simulink library "ammclib_bam_S32K3xx"  (R2016a)
settings: Solver=VariableStepAuto  SolverMode=SingleTasking  StartTime=0.0  StopTime=10.0  RelTol=1e-3
undefined symbols (not defined in the file or in its folder): a1, a2, ADCMaxError, autoCalcEn, b0, b1, b2, cfg, dgain, escale, f16A1, f16A2, f16ADCMaxError, f16B0, f16B1, f16B2, f16C1, f16CC1sc, f16CC1sc_D, f16CC1sc_Q, f16CC2sc, f16CC2sc_D, f16CC2sc_Q, f16DerivGain, f16EGain, f16FiltCoef, f16HystOff, f16HystOn, f16IGain, f16IntegGain, f16IntegGain_D, f16IntegGain_Q, f16IntegGainQ, f16Kd, f16KLs, f16Kq, f16KRs, f16Limit, f16LowerLimit, f16LowerLimit_D, f16LowerLimit_Q, f16LowerLimitQ, f16ModIndex, f16OutValOff, f16OutValOn, f16PropGain, f16PropGain_D, f16PropGain_Q, f16PropGainQ, f16RampDown, f16RampUp, f16UGain, f16UpperLimit, f16UpperLimit_D, f16UpperLimit_Q, f16UpperLimitQ, f16WIGain, f32A1, f32A2, f32ADCMaxError ... (+180)
(part 39 of 50)

== system ammclib_bam_S32K3xx/GFLIB/FLT ==
  GFLIB_Acos_FLT : Subsystem  TreatAsAtomicUnit=on  mask(GFLIB_Acos_FLT){}
      mask help: Inverse cosine function in single precision floating-point implementation. Refer to the AMMCLIB User's Guide for further details.
      mask init: same as ammclib_bam_S32K3xx/GDFLIB/F16/GDFLIB_FilterFIR_F16
      settings: RTWSystemCode=Inline
      mask Help: web([fileparts(which('ammclib_bam_S32K3xx.slx')) '/../doc/S32K3XXMCLUG.pdf'], '-browser')
      mask Display: pos = get_param(gcb, 'Position');width = pos(3) - pos(1); height = pos(4) - pos(2);tX=width/2;tY=height - 8;color('black');text(tX,tY, 'GFLIB_Acos_FLT', 'horizontalAlignment', 'center');
  GFLIB_Asin_FLT : Subsystem  TreatAsAtomicUnit=on  mask(GFLIB_Asin_FLT){}
      mask help: Inverse sine function in single precision floating-point implementation. Refer to the AMMCLIB User's Guide for further details.
      mask init: same as ammclib_bam_S32K3xx/GDFLIB/F16/GDFLIB_FilterFIR_F16
      settings: RTWSystemCode=Inline
      mask Help: web([fileparts(which('ammclib_bam_S32K3xx.slx')) '/../doc/S32K3XXMCLUG.pdf'], '-browser')
      mask Display: pos = get_param(gcb, 'Position');width = pos(3) - pos(1); height = pos(4) - pos(2);tX=width/2;tY=height - 8;color('black');text(tX,tY, 'GFLIB_Asin_FLT', 'horizontalAlignment', 'center');
  GFLIB_AtanYXShifted_FLT : Subsystem  TreatAsAtomicUnit=on  mask(GFLIB_AtanYXShifted_FLT){}
      mask help: Shifted arctangent of two arguments Y/X in single precision floating-point implementation. Refer to the AMMCLIB User's Guide for further details.
      mask init: same as ammclib_bam_S32K3xx/GDFLIB/F16/GDFLIB_FilterFIR_F16
      settings: RTWSystemCode=Inline
      mask Help: web([fileparts(which('ammclib_bam_S32K3xx.slx')) '/../doc/S32K3XXMCLUG.pdf'], '-browser')
      mask Display: pos = get_param(gcb, 'Position');width = pos(3) - pos(1); height = pos(4) - pos(2);tX=width/2;tY=height - 8;color('black');text(tX,tY, 'GFLIB_AtanYXShifted_FLT', 'horizontalAlignment', 'center');
  GFLIB_AtanYX_FLT : Subsystem  TreatAsAtomicUnit=on  mask(GFLIB_AtanYX_FLT){}
      mask help: Arctangent of two arguments Y/X in single precision floating-point implementation. Refer to the AMMCLIB User's Guide for further details.
      mask init: same as ammclib_bam_S32K3xx/GDFLIB/F16/GDFLIB_FilterFIR_F16
      settings: RTWSystemCode=Inline
      mask Help: web([fileparts(which('ammclib_bam_S32K3xx.slx')) '/../doc/S32K3XXMCLUG.pdf'], '-browser')
      mask Display: pos = get_param(gcb, 'Position');width = pos(3) - pos(1); height = pos(4) - pos(2);tX=width/2;tY=height - 8;color('black');text(tX,tY, 'GFLIB_AtanYX_FLT', 'horizontalAlignment', 'center');
  GFLIB_Atan_FLT : Subsystem  TreatAsAtomicUnit=on  mask(GFLIB_Atan_FLT){}
      mask help: Inverse tangent function in single precision floating-point implementation. Refer to the AMMCLIB User's Guide for further details.
      mask init: same as ammclib_bam_S32K3xx/GDFLIB/F16/GDFLIB_FilterFIR_F16
      settings: RTWSystemCode=Inline
      mask Help: web([fileparts(which('ammclib_bam_S32K3xx.slx')) '/../doc/S32K3XXMCLUG.pdf'], '-browser')
      mask Display: pos = get_param(gcb, 'Position');width = pos(3) - pos(1); height = pos(4) - pos(2);tX=width/2;tY=height - 8;color('black');text(tX,tY, 'GFLIB_Atan_FLT', 'horizontalAlignment', 'center');
  GFLIB_ControllerPIDpAW_FLT : Subsystem  StartFcn=|  TreatAsAtomicUnit=on  mask(GFLIB_ControllerPIDpAW_FLT){showStates=Hide (faster execution), resetStatesEnable=Pre-set according to the first set of inputs after reset, SampleTime=-1, pgain=5, igain=0.5, dgain=0.01, filtCoef=10, lowerLimit=-10, upperLimit=10, autoCalcEn=on, fltPropGain=0, fltIntegGain=0, fltDerivGain=0, fltFiltCoef=0, fltLowerLimit=0, fltUpperLimit=0, SampleTime_1=NaN}
      | ts=get_param(gcb,'CompiledSampleTime');
      | if iscell(ts)
      |   ts=ts{1};
      |   if iscell(ts)
      |     ts=ts{1};
      |   end
      | end
      | ts=ts(1);
      | set_param(gcb,'SampleTime_1',num2str(ts));
      | p=Simulink.Mask.get(gcb);
      | hintText=p.getDialogControl('timeHint');
      | SampleTime=Simulink.data.evalinGlobal(bdroot,get_param(gcb,'SampleTime'));
      | p=Simulink.Mask.get(gcb);
      | autoCalcEn=get_param(gcb,'autoCalcEn');
      | if strcmp(autoCalcEn,'on')
      |   if SampleTime==-1
      |     hintText.Prompt='Caution: Implementation parameters depend on inherited sample time. Make sure that the sample time of the block''s inputs corresponds to the sampling period in the target application.';
      |   else
      |     hintText.Prompt='Caution: Implementation parameters depend on the sample time. Make sure that the simulation time step corresponds to the sampling period in the target application.';
      |   end
      |   SampleTime=ts;
      |   fltPropGain_bkup=get_param(gcb,'fltPropGain');
      |   fltIntegGain_bkup=get_param(gcb,'fltIntegGain');
      |   fltDerivGain_bkup=get_param(gcb,'fltDerivGain');
      |   fltFiltCoef_bkup=get_param(gcb,'fltFiltCoef');
      |   fltLowerLimit_bkup=get_param(gcb,'fltLowerLimit');
      |   fltUpperLimit_bkup=get_param(gcb,'fltUpperLimit');
      |   pgain=Simulink.data.evalinGlobal(bdroot,get_param(gcb,'pgain'));
      |   igain=Simulink.data.evalinGlobal(bdroot,get_param(gcb,'igain'));
      |   dgain=Simulink.data.evalinGlobal(bdroot,get_param(gcb,'dgain'));
      |   filtCoef=Simulink.data.evalinGlobal(bdroot,get_param(gcb,'filtCoef'));
      |   lowerLimit=Simulink.data.evalinGlobal(bdroot,get_param(gcb,'lowerLimit'));
      |   upperLimit=Simulink.data.evalinGlobal(bdroot,get_param(gcb,'upperLimit'));
      |   if (upperLimit<=lowerLimit)
      |     warning('UpperLimit should be greater than LowerLimit.');
      |   end
      |   fltPropGain=pgain;
      |   fltIntegGain=igain*SampleTime*0.5;
      |   exparg=-SampleTime*filtCoef;
      |   expconst=exp(exparg);
      |   fltFiltCoef=expconst;
      |   fltDerivGain=dgain/SampleTime*(1 - expconst);
      |   fltUpperLimit=upperLimit;
      |   fltLowerLimit=lowerLimit;
      |   if isnan(fltPropGain)
      |     if ~strcmp(fltPropGain_bkup,'0')
      |       set_param(gcb,'fltPropGain','0');
      |     end
      |   else
      |     tmps=num2str(fltPropGain);
      |     if ~strcmp(fltPropGain_bkup,tmps)
      |       set_param(gcb,'fltPropGain',tmps);
      |     end
      |   end
      |   if isnan(fltIntegGain)
      |     if ~strcmp(fltIntegGain_bkup,'0')
      |       set_param(gcb,'fltIntegGain','0');
      |     end
      |   else
      |     tmps=num2str(fltIntegGain);
      |     if ~strcmp(fltIntegGain_bkup,tmps)
      |       set_param(gcb,'fltIntegGain',tmps);
      |     end
      |   end
      |   if isnan(fltDerivGain)
      |     if ~strcmp(fltDerivGain_bkup,'0')
      |       set_param(gcb,'fltDerivGain','0');
      |     end
      |   else
      |     tmps=num2str(fltDerivGain);
      |     if ~strcmp(fltDerivGain_bkup,tmps)
      |       set_param(gcb,'fltDerivGain',tmps);
      |     end
      |   end
      |   if isnan(fltFiltCoef)
      |     if ~strcmp(fltFiltCoef_bkup,'0')
      |       set_param(gcb,'fltFiltCoef','0');
      |     end
      |   else
      |     tmps=num2str(fltFiltCoef);
      |     if ~strcmp(fltFiltCoef_bkup,tmps)
      |       set_param(gcb,'fltFiltCoef',tmps);
      |     end
      |   end
      |   if isnan(fltLowerLimit)
      |     if ~strcmp(fltLowerLimit_bkup,'0')
      |       set_param(gcb,'fltLowerLimit','0');
      |     end
      |   else
      |     tmps=num2str(fltLowerLimit);
      |     if ~strcmp(fltLowerLimit_bkup,tmps)
      |       set_param(gcb,'fltLowerLimit',tmps);
      |     end
      |   end
      |   if isnan(fltUpperLimit)
      |     if ~strcmp(fltUpperLimit_bkup,'0')
      |       set_param(gcb,'fltUpperLimit','0');
      |     end
      |   else
      |     tmps=num2str(fltUpperLimit);
      |     if ~strcmp(fltUpperLimit_bkup,tmps)
      |       set_param(gcb,'fltUpperLimit',tmps);
      |     end
      |   end
      | end
      mask prompts: showStates "Show internal states:"; resetStatesEnable "Internal state after reset:"; SampleTime "Sample time (-1 for inherited):"; pgain "Proportional gain (P):"; igain "Integral gain (I):"; dgain "Derivative gain (D):"; filtCoef "Derivative gain limit N (usually 3 to 20):"; lowerLimit "Controller lower limit:"; upperLimit "Controller upper limit:"; autoCalcEn "Calculate implementation parameters from physical parameters"; fltPropGain "fltPropGain (Proportional gain):"; fltIntegGain "fltIntegGain (Integral gain):"; fltDerivGain "fltDerivGain (Derivative Gain):"; fltFiltCoef "fltFiltCoef (Derivative term filter coefficient):"; fltLowerLimit "fltLowerLimit (Lower Limit of the controller):"; fltUpperLimit "fltUpperLimit (Upper Limit of the controller):"; SampleTime_1 "Discrete sample time:"
      mask help: Parallel form of a discrete-time PID controller with anti-windup in single precision floating-point implementation. This block supports re-initialization of the internal state during simulation. If the block is reset, the controller's output will be aligned with the input fltControllerPIDpAWOut_preset. Refer to the AMMCLIB User's Guide for further details.
      mask init:
      | ddName = get_param(bdroot,'DataDictionary');
      | if length(ddName)==0
      |   set_param(bdroot,'DataDictionary','ammclib_types.sldd');
      | else
      |   dd = Simulink.data.dictionary.open(ddName);
      |   data = getSection(dd,'Design Data');
      |   if ~exist(data,'SWLIBS_2Syst_F16')
      |     addDataSource(dd,'ammclib_types.sldd');
      |     saveChanges(dd);
      |   end
      | end
      | 
      | if showStates == 1
      |   % hidden state variables
      |   if strcmp(get_param([gcb '/fltPropGain'], 'BlockType'), 'Inport')
      |     posblk = get_param(gcb, 'Position');
      | 
      |     pos = get_param([gcb, '/fltPropGain'], 'Position');
      |     orient = get_param([gcb, '/fltPropGain'], 'Orientation');
      |     delete_block([gcb, '/fltPropGain']);
      |     add_block('built-in/Ground', [gcb, '/fltPropGain'], 'Position', pos, 'Orientation', orient);
      | 
      |     pos = get_param([gcb, '/fltIntegGain'], 'Position');
      |     orient = get_param([gcb, '/fltIntegGain'], 'Orientation');
      |     delete_block([gcb, '/fltIntegGain']);
      |     add_block('built-in/Ground', [gcb, '/fltIntegGain'], 'Position', pos, 'Orientation', orient);
      | 
      |     pos = get_param([gcb, '/fltDerivGain'], 'Position');
      |     orient = get_param([gcb, '/fltDerivGain'], 'Orientation');
      |     delete_block([gcb, '/fltDerivGain']);
      |     add_block('built-in/Ground', [gcb, '/fltDerivGain'], 'Position', pos, 'Orientation', orient);
      | 
      |     pos = get_param([gcb, '/fltFiltCoef'], 'Position');
      |     orient = get_param([gcb, '/fltFiltCoef'], 'Orientation');
      |     delete_block([gcb, '/fltFiltCoef']);
      |     add_block('built-in/Ground', [gcb, '/fltFiltCoef'], 'Position', pos, 'Orientation', orient);
      | 
      |     pos = get_param([gcb, '/fltLowerLimit'], 'Position');
      |     orient = get_param([gcb, '/fltLowerLimit'], 'Orientation');
      |     delete_block([gcb, '/fltLowerLimit']);
      |     add_block('built-in/Ground', [gcb, '/fltLowerLimit'], 'Position', pos, 'Orientation', orient);
      | 
      |     pos = get_param([gcb, '/fltUpperLimit'], 'Position');
      |     orient = get_param([gcb, '/fltUpperLimit'], 'Orientation');
      |     delete_block([gcb, '/fltUpperLimit']);
      |     add_block('built-in/Ground', [gcb, '/fltUpperLimit'], 'Position', pos, 'Orientation', orient);
      | 
      |     pos = get_param([gcb, '/fltIntegPartK_1'], 'Position');
      |     orient = get_param([gcb, '/fltIntegPartK_1'], 'Orientation');
      |     delete_block([gcb, '/fltIntegPartK_1']);
      |     add_block('built-in/Ground', [gcb, '/fltIntegPartK_1'], 'Position', pos, 'Orientation', orient);
      | 
      |     pos = get_param([gcb, '/fltDerivPartK_1'], 'Position');
      |     orient = get_param([gcb, '/fltDerivPartK_1'], 'Orientation');
      |     delete_block([gcb, '/fltDerivPartK_1']);
      |     add_block('built-in/Ground', [gcb, '/fltDerivPartK_1'], 'Position', pos, 'Orientation', orient);
      | 
      |     pos = get_param([gcb, '/fltInK_1'], 'Position');
      |     orient = get_param([gcb, '/fltInK_1'], 'Orientation');
      |     delete_block([gcb, '/fltInK_1']);
      |     add_block('built-in/Ground', [gcb, '/fltInK_1'], 'Position', pos, 'Orientation', orient);
      | 
      | 
      |     pmask=Simulink.Mask.get(gcb);
      |     pctrl=pmask.getParameter('SampleTime');
      |     pctrl.set('TypeOptions',{'fltInErr/SampleTime','fltControllerPIDpAWOut_preset/SampleTime'});
      | 
      |     pos = get_param([gcb '/fltIntegPartK_1_Out'], 'Position');
      |     orient = get_param([gcb '/fltIntegPartK_1_Out'], 'Orientation');
      |     delete_block([gcb '/fltIntegPartK_1_Out']);
      |     add_block('built-in/Terminator', [gcb '/fltIntegPartK_1_Out'], 'Position', pos, 'Orientation', orient);
      | 
      |     pos = get_param([gcb '/fltDerivPartK_1_Out'], 'Position');
      |     orient = get_param([gcb '/fltDerivPartK_1_Out'], 'Orientation');
      |     delete_block([gcb '/fltDerivPartK_1_Out']);
      |     add_block('built-in/Terminator', [gcb '/fltDerivPartK_1_Out'], 'Position', pos, 'Orientation', orient);
      | 
      |     pos = get_param([gcb '/fltInK_1_Out'], 'Position');
      |     orient = get_param([gcb '/fltInK_1_Out'], 'Orientation');
      |     delete_block([gcb '/fltInK_1_Out']);
      |     add_block('built-in/Terminator', [gcb '/fltInK_1_Out'], 'Position', pos, 'Orientation', orient);
      | 
      |     set_param([gcb '/fltInErr'], 'Port', '1');
      |     set_param([gcb '/fltControllerPIDpAWOut_preset'], 'Port', '2');
      | 
      |     tmpOutCnt=0;
      |     tmpOutCnt=tmpOutCnt+1;
      |     set_param([gcb '/fltOut'], 'Port', num2str(tmpOutCnt));
      |     tmpOutCnt=tmpOutCnt+1;
      |     set_param([gcb '/u16LimitFlag'], 'Port', num2str(tmpOutCnt));
      | 
      |     autoCalcEn=get_param(gcb,'autoCalcEn');
      |     if strcmp(autoCalcEn,'on')
      |       set_param(gcb,'MaskEnables',{'on','on','on','on','on','on','on','on','on','on','on','on','on','on','on','on','off'});
      |     else
      |       set_param(gcb,'MaskEnables',{'on','on','on','off','off','off','off','off','off','on','on','on','on','on','on','on','off'});
      |     end
      | 
      |     if (posblk(4) - posblk(2)) > 75
      |       height = 75;
      |       set_param(gcb,'Position',[posblk(1), posblk(2), posblk(3), posblk(2)+height])
      |     end
      |   end
      | else
      |   % shown state variables
      |   if strcmp(get_param([gcb '/fltPropGain'], 'BlockType'), 'Ground')
      |     posblk = get_param(gcb, 'Position');
      | 
      |     pos = get_param([gcb, '/fltPropGain'], 'Position');
      |     orient = get_param([gcb, '/fltPropGain'], 'Orientation');
      |     delete_block([gcb, '/fltPropGain']);
      |     add_block('built-in/Inport', [gcb, '/fltPropGain'], 'Position', pos, 'Orientation', orient, 'OutDataTypeStr', 'single');
      | 
      |     pos = get_param([gcb, '/fltIntegGain'], 'Position');
      |     orient = get_param([gcb, '/fltIntegGain'], 'Orientation');
      |     delete_block([gcb, '/fltIntegGain']);
      |     add_block('built-in/Inport', [gcb, '/fltIntegGain'], 'Position', pos, 'Orientation', orient, 'OutDataTypeStr', 'single');
      | 
      |     pos = get_param([gcb, '/fltDerivGain'], 'Position');
      |     orient = get_param([gcb, '/fltDerivGain'], 'Orientation');
      |     delete_block([gcb, '/fltDerivGain']);
      |     add_block('built-in/Inport', [gcb, '/fltDerivGain'], 'Position', pos, 'Orientation', orient, 'OutDataTypeStr', 'single');
      | 
      |     pos = get_param([gcb, '/fltFiltCoef'], 'Position');
      |     orient = get_param([gcb, '/fltFiltCoef'], 'Orientation');
      |     delete_block([gcb, '/fltFiltCoef']);
      |     add_block('built-in/Inport', [gcb, '/fltFiltCoef'], 'Position', pos, 'Orientation', orient, 'OutDataTypeStr', 'single');
      | 
      |     pos = get_param([gcb, '/fltLowerLimit'], 'Position');
      |     orient = get_param([gcb, '/fltLowerLimit'], 'Orientation');
      |     delete_block([gcb, '/fltLowerLimit']);
      |     add_block('built-in/Inport', [gcb, '/fltLowerLimit'], 'Position', pos, 'Orientation', orient, 'OutDataTypeStr', 'single');
      | 
      |     pos = get_param([gcb, '/fltUpperLimit'], 'Position');
      |     orient = get_param([gcb, '/fltUpperLimit'], 'Orientation');
      |     delete_block([gcb, '/fltUpperLimit']);
      |     add_block('built-in/Inport', [gcb, '/fltUpperLimit'], 'Position', pos, 'Orientation', orient, 'OutDataTypeStr', 'single');
      | 
      |     pos = get_param([gcb, '/fltIntegPartK_1'], 'Position');
      |     orient = get_param([gcb, '/fltIntegPartK_1'], 'Orientation');
      |     delete_block([gcb, '/fltIntegPartK_1']);
      |     add_block('built-in/Inport', [gcb, '/fltIntegPartK_1'], 'Position', pos, 'Orientation', orient, 'OutDataTypeStr', 'single');
      | 
      |     pos = get_param([gcb, '/fltDerivPartK_1'], 'Position');
      |     orient = get_param([gcb, '/fltDerivPartK_1'], 'Orientation');
      |     delete_block([gcb, '/fltDerivPartK_1']);
      |     add_block('built-in/Inport', [gcb, '/fltDerivPartK_1'], 'Position', pos, 'Orientation', orient, 'OutDataTypeStr', 'single');
      | 
      |     pos = get_param([gcb, '/fltInK_1'], 'Position');
      |     orient = get_param([gcb, '/fltInK_1'], 'Orientation');
      |     delete_block([gcb, '/fltInK_1']);
      |     add_block('built-in/Inport', [gcb, '/fltInK_1'], 'Position', pos, 'Orientation', orient, 'OutDataTypeStr', 'single');
      | 
      | 
      | 
      |     pos = get_param([gcb '/fltIntegPartK_1_Out'], 'Position');
      |     orient = get_param([gcb '/fltIntegPartK_1_Out'], 'Orientation');
      |     delete_block([gcb '/fltIntegPartK_1_Out']);
      |     add_block('built-in/Outport', [gcb '/fltIntegPartK_1_Out'], 'Position', pos, 'Orientation', orient);
      | 
      |     pos = get_param([gcb '/fltDerivPartK_1_Out'], 'Position');
      |     orient = get_param([gcb '/fltDerivPartK_1_Out'], 'Orientation');
      |     delete_block([gcb '/fltDerivPartK_1_Out']);
      |     add_block('built-in/Outport', [gcb '/fltDerivPartK_1_Out'], 'Position', pos, 'Orientation', orient);
      | 
      |     pos = get_param([gcb '/fltInK_1_Out'], 'Position');
      |     orient = get_param([gcb '/fltInK_1_Out'], 'Orientation');
      |     delete_block([gcb '/fltInK_1_Out']);
      |     add_block('built-in/Outport', [gcb '/fltInK_1_Out'], 'Position', pos, 'Orientation', orient);
      | 
      | 
      |     pmask=Simulink.Mask.get(gcb);
      |     pctrl=pmask.getParameter('SampleTime');
      |     pctrl.set('TypeOptions',{'fltInErr/SampleTime','fltControllerPIDpAWOut_preset/SampleTime','fltPropGain/SampleTime','fltIntegGain/SampleTime','fltDerivGain/SampleTime','fltFiltCoef/SampleTime','fltLowerLimit/SampleTime','fltUpperLimit/SampleTime','fltIntegPartK_1/SampleTime','fltDerivPartK_1/SampleTime','fltInK_1/SampleTime'});
      | 
      |     set_param([gcb '/fltInErr'], 'Port', '1');
      |     set_param([gcb '/fltControllerPIDpAWOut_preset'], 'Port', '2');
      |     set_param([gcb '/fltPropGain'], 'Port', '3');
      |     set_param([gcb '/fltIntegGain'], 'Port', '4');
      |     set_param([gcb '/fltDerivGain'], 'Port', '5');
      |     set_param([gcb '/fltFiltCoef'], 'Port', '6');
      |     set_param([gcb '/fltLowerLimit'], 'Port', '7');
      |     set_param([gcb '/fltUpperLimit'], 'Port', '8');
      |     set_param([gcb '/fltIntegPartK_1'], 'Port', '9');
      |     set_param([gcb '/fltDerivPartK_1'], 'Port', '10');
      |     set_param([gcb '/fltInK_1'], 'Port', '11');
      | 
      |     tmpOutCnt=0;
      |     tmpOutCnt=tmpOutCnt+1;
      |     set_param([gcb '/fltOut'], 'Port', num2str(tmpOutCnt));
      |     tmpOutCnt=tmpOutCnt+1;
      |     set_param([gcb '/u16LimitFlag'], 'Port', num2str(tmpOutCnt));
      |     tmpOutCnt=tmpOutCnt+1;
      |     set_param([gcb '/fltIntegPartK_1_Out'], 'Port', num2str(tmpOutCnt));
      |     tmpOutCnt=tmpOutCnt+1;
      |     set_param([gcb '/fltDerivPartK_1_Out'], 'Port', num2str(tmpOutCnt));
      |     tmpOutCnt=tmpOutCnt+1;
      |     set_param([gcb '/fltInK_1_Out'], 'Port', num2str(tmpOutCnt));
      | 
      |     set_param(gcb,'MaskEnables',{'on','on','on','off','off','off','off','off','off','off','off','off','off','off','off','off','off'});
      | 
      |     if (posblk(4) - posblk(2)) < 300
      |       height = 300;
      |       set_param(gcb,'Position',[posblk(1), posblk(2), posblk(3), posblk(2)+height])
      |     end
      |   end
      | end
      settings: RTWSystemCode=Inline
      mask Help: web([fileparts(which('ammclib_bam_S32K3xx.slx')) '/../doc/S32K3XXMCLUG.pdf'], '-browser')
      mask TypeOptions showStates: Hide (faster execution) | Show (allows debugging; connect feedback loops manually)
      mask Callback showStates:
      | maskStr=get_param(gcb,'showStates');
      | if strcmp(maskStr,'Hide (faster execution)')
      |   if strcmp(get_param([gcb '/fltPropGain'], 'BlockType'), 'Inport')
      |     autoCalcEn=get_param(gcb,'autoCalcEn');
      |     if strcmp(autoCalcEn,'on')
      |       set_param(gcb,'MaskEnables',{'on','on','on','on','on','on','on','on','on','on','on','on','on','on','on','on','off'});
      |     else
      |       set_param(gcb,'MaskEnables',{'on','on','on','off','off','off','off','off','off','on','on','on','on','on','on','on','off'});
      |     end
      |   end
      | else
      |   if strcmp(get_param([gcb '/fltPropGain'], 'BlockType'), 'Ground')
      |     set_param(gcb,'MaskEnables',{'on','on','on','off','off','off','off','off','off','off','off','off','off','off','off','off','off'});
      |   end
      | end
      mask TypeOptions resetStatesEnable: Pre-set according to the first set of inputs after reset | Clear to zero
      mask TypeOptions SampleTime: fltInErr/SampleTime | fltControllerPIDpAWOut_preset/SampleTime
      mask Callback SampleTime:
      | p=Simulink.Mask.get(gcb);
      | hintText=p.getDialogControl('timeHint');
      | SampleTime=Simulink.data.evalinGlobal(bdroot,get_param(gcb,'SampleTime'));
      | SampleTime_1=str2double(get_param(gcb,'SampleTime_1'));
      | if (((SampleTime==-1) && (~contains(hintText.Prompt,'inherited'))) || ...
      |     ((SampleTime~=-1) && contains(hintText.Prompt,'inherited')) || ...
      |     ((SampleTime~=-1) && (SampleTime_1~=SampleTime)) || ...
      |     ((SampleTime_1~=-1) && contains(hintText.Prompt,'yet')))
      |   if ((SampleTime==-1) && (~contains(hintText.Prompt,'inherited')))
      |     set_param(gcb,'SampleTime_1',num2str(NaN));
      |     SampleTime_1=NaN;
      |   end
      |   if (SampleTime~=-1)
      |     set_param(gcb,'SampleTime_1',num2str(SampleTime));
      |     SampleTime_1=SampleTime;
      |   end
      |   autoCalcEn=get_param(gcb,'autoCalcEn');
      |   if strcmp(autoCalcEn,'on')
      |     p=Simulink.Mask.get(gcb);
      |     hintText=p.getDialogControl('timeHint');
      |     if SampleTime==-1
      |       SampleTime=SampleTime_1;
      |       if isnan(SampleTime)
      |         hintText.Prompt='Note: Implementation parameters cannot be calculated yet because the block''s inherited sample time is unknown. Simulink will update the sample time when you run the simulation.';
      |       else
      |         hintText.Prompt='Caution: Implementation parameters depend on inherited sample time. Make sure that the sample time of the block''s inputs corresponds to the sampling period in the target application.';
      |       end
      |     else
      |       hintText.Prompt='Caution: Implementation parameters depend on the sample time. Make sure that the simulation time step corresponds to the sampling period in the target application.';
      |     end
      |     fltPropGain_bkup=get_param(gcb,'fltPropGain');
      |     fltIntegGain_bkup=get_param(gcb,'fltIntegGain');
      |     fltDerivGain_bkup=get_param(gcb,'fltDerivGain');
      |     fltFiltCoef_bkup=get_param(gcb,'fltFiltCoef');
      |     fltLowerLimit_bkup=get_param(gcb,'fltLowerLimit');
      |     fltUpperLimit_bkup=get_param(gcb,'fltUpperLimit');
      |     pgain=Simulink.data.evalinGlobal(bdroot,get_param(gcb,'pgain'));
      |     igain=Simulink.data.evalinGlobal(bdroot,get_param(gcb,'igain'));
      |     dgain=Simulink.data.evalinGlobal(bdroot,get_param(gcb,'dgain'));
      |     filtCoef=Simulink.data.evalinGlobal(bdroot,get_param(gcb,'filtCoef'));
      |     lowerLimit=Simulink.data.evalinGlobal(bdroot,get_param(gcb,'lowerLimit'));
      |     upperLimit=Simulink.data.evalinGlobal(bdroot,get_param(gcb,'upperLimit'));
      |     if (upperLimit<=lowerLimit)
      |       warning('UpperLimit should be greater than LowerLimit.');
      |     end
      |     fltPropGain=pgain;
      |     fltIntegGain=igain*SampleTime*0.5;
      |     exparg=-SampleTime*filtCoef;
      |     expconst=exp(exparg);
      |     fltFiltCoef=expconst;
      |     fltDerivGain=dgain/SampleTime*(1 - expconst);
      |     fltUpperLimit=upperLimit;
      |     fltLowerLimit=lowerLimit;
      |     if isnan(fltPropGain)
      |       if ~strcmp(fltPropGain_bkup,'0')
      |         set_param(gcb,'fltPropGain','0');
      |       end
      |     else
      |       tmps=num2str(fltPropGain);
      |       if ~strcmp(fltPropGain_bkup,tmps)
      |         set_param(gcb,'fltPropGain',tmps);
      |       end
      |     end
      |     if isnan(fltIntegGain)
      |       if ~strcmp(fltIntegGain_bkup,'0')
      |         set_param(gcb,'fltIntegGain','0');
      |       end
      |     else
      |       tmps=num2str(fltIntegGain);
      |       if ~strcmp(fltIntegGain_bkup,tmps)
      |         set_param(gcb,'fltIntegGain',tmps);
      |       end
      |     end
      |     if isnan(fltDerivGain)
      |       if ~strcmp(fltDerivGain_bkup,'0')
      |         set_param(gcb,'fltDerivGain','0');
      |       end
      |     else
      |       tmps=num2str(fltDerivGain);
      |       if ~strcmp(fltDerivGain_bkup,tmps)
      |         set_param(gcb,'fltDerivGain',tmps);
      |       end
      |     end
      |     if isnan(fltFiltCoef)
      |       if ~strcmp(fltFiltCoef_bkup,'0')
      |         set_param(gcb,'fltFiltCoef','0');
      |       end
      |     else
      |       tmps=num2str(fltFiltCoef);
      |       if ~strcmp(fltFiltCoef_bkup,tmps)
      |         set_param(gcb,'fltFiltCoef',tmps);
      |       end
      |     end
      |     if isnan(fltLowerLimit)
      |       if ~strcmp(fltLowerLimit_bkup,'0')
      |         set_param(gcb,'fltLowerLimit','0');
      |       end
      |     else
      |       tmps=num2str(fltLowerLimit);
      |       if ~strcmp(fltLowerLimit_bkup,tmps)
      |         set_param(gcb,'fltLowerLimit',tmps);
      |       end
      |     end
      |     if isnan(fltUpperLimit)
      |       if ~strcmp(fltUpperLimit_bkup,'0')
      |         set_param(gcb,'fltUpperLimit','0');
      |       end
      |     else
      |       tmps=num2str(fltUpperLimit);
      |       if ~strcmp(fltUpperLimit_bkup,tmps)
      |         set_param(gcb,'fltUpperLimit',tmps);
      |       end
      |     end
      |   end
      | end
      mask Callback pgain:
      | autoCalcEn=get_param(gcb,'autoCalcEn');
      | if strcmp(autoCalcEn,'on')
      |   SampleTime=Simulink.data.evalinGlobal(bdroot,get_param(gcb,'SampleTime'));
      |   if (SampleTime==-1)
      |     SampleTime=str2double(get_param(gcb,'SampleTime_1'));
      |   end
      |   fltPropGain_bkup=get_param(gcb,'fltPropGain');
      |   fltIntegGain_bkup=get_param(gcb,'fltIntegGain');
      |   fltDerivGain_bkup=get_param(gcb,'fltDerivGain');
      |   fltFiltCoef_bkup=get_param(gcb,'fltFiltCoef');
      |   fltLowerLimit_bkup=get_param(gcb,'fltLowerLimit');
      |   fltUpperLimit_bkup=get_param(gcb,'fltUpperLimit');
      |   pgain=Simulink.data.evalinGlobal(bdroot,get_param(gcb,'pgain'));
      |   igain=Simulink.data.evalinGlobal(bdroot,get_param(gcb,'igain'));
      |   dgain=Simulink.data.evalinGlobal(bdroot,get_param(gcb,'dgain'));
      |   filtCoef=Simulink.data.evalinGlobal(bdroot,get_param(gcb,'filtCoef'));
      |   lowerLimit=Simulink.data.evalinGlobal(bdroot,get_param(gcb,'lowerLimit'));
      |   upperLimit=Simulink.data.evalinGlobal(bdroot,get_param(gcb,'upperLimit'));
      |   if (upperLimit<=lowerLimit)
      |     warning('UpperLimit should be greater than LowerLimit.');
      |   end
      |   fltPropGain=pgain;
      |   fltIntegGain=igain*SampleTime*0.5;
      |   exparg=-SampleTime*filtCoef;
      |   expconst=exp(exparg);
      |   fltFiltCoef=expconst;
      |   fltDerivGain=dgain/SampleTime*(1 - expconst);
      |   fltUpperLimit=upperLimit;
      |   fltLowerLimit=lowerLimit;
      |   if isnan(fltPropGain)
      |     if ~strcmp(fltPropGain_bkup,'0')
      |       set_param(gcb,'fltPropGain','0');
      |     end
      |   else
      |     tmps=num2str(fltPropGain);
      |     if ~strcmp(fltPropGain_bkup,tmps)
      |       set_param(gcb,'fltPropGain',tmps);
      |     end
      |   end
      |   if isnan(fltIntegGain)
      |     if ~strcmp(fltIntegGain_bkup,'0')
      |       set_param(gcb,'fltIntegGain','0');
      |     end
      |   else
      |     tmps=num2str(fltIntegGain);
      |     if ~strcmp(fltIntegGain_bkup,tmps)
      |       set_param(gcb,'fltIntegGain',tmps);
      |     end
      |   end
      |   if isnan(fltDerivGain)
      |     if ~strcmp(fltDerivGain_bkup,'0')
      |       set_param(gcb,'fltDerivGain','0');
      |     end
      |   else
      |     tmps=num2str(fltDerivGain);
      |     if ~strcmp(fltDerivGain_bkup,tmps)
      |       set_param(gcb,'fltDerivGain',tmps);
      |     end
      |   end
      |   if isnan(fltFiltCoef)
      |     if ~strcmp(fltFiltCoef_bkup,'0')
      |       set_param(gcb,'fltFiltCoef','0');
      |     end
      |   else
      |     tmps=num2str(fltFiltCoef);
      |     if ~strcmp(fltFiltCoef_bkup,tmps)
      |       set_param(gcb,'fltFiltCoef',tmps);
      |     end
      |   end
      |   if isnan(fltLowerLimit)
      |     if ~strcmp(fltLowerLimit_bkup,'0')
      |       set_param(gcb,'fltLowerLimit','0');
      |     end
      |   else
      |     tmps=num2str(fltLowerLimit);
      |     if ~strcmp(fltLowerLimit_bkup,tmps)
      |       set_param(gcb,'fltLowerLimit',tmps);
      |     end
      |   end
      |   if isnan(fltUpperLimit)
      |     if ~strcmp(fltUpperLimit_bkup,'0')
      |       set_param(gcb,'fltUpperLimit','0');
      |     end
      |   else
      |     tmps=num2str(fltUpperLimit);
      |     if ~strcmp(fltUpperLimit_bkup,tmps)
      |       set_param(gcb,'fltUpperLimit',tmps);
      |     end
      |   end
      | end
      mask Callback igain:
      | autoCalcEn=get_param(gcb,'autoCalcEn');
      | if strcmp(autoCalcEn,'on')
      |   SampleTime=Simulink.data.evalinGlobal(bdroot,get_param(gcb,'SampleTime'));
      |   if (SampleTime==-1)
      |     SampleTime=str2double(get_param(gcb,'SampleTime_1'));
      |   end
      |   fltPropGain_bkup=get_param(gcb,'fltPropGain');
      |   fltIntegGain_bkup=get_param(gcb,'fltIntegGain');
      |   fltDerivGain_bkup=get_param(gcb,'fltDerivGain');
      |   fltFiltCoef_bkup=get_param(gcb,'fltFiltCoef');
      |   fltLowerLimit_bkup=get_param(gcb,'fltLowerLimit');
      |   fltUpperLimit_bkup=get_param(gcb,'fltUpperLimit');
      |   pgain=Simulink.data.evalinGlobal(bdroot,get_param(gcb,'pgain'));
      |   igain=Simulink.data.evalinGlobal(bdroot,get_param(gcb,'igain'));
      |   dgain=Simulink.data.evalinGlobal(bdroot,get_param(gcb,'dgain'));
      |   filtCoef=Simulink.data.evalinGlobal(bdroot,get_param(gcb,'filtCoef'));
      |   lowerLimit=Simulink.data.evalinGlobal(bdroot,get_param(gcb,'lowerLimit'));
      |   upperLimit=Simulink.data.evalinGlobal(bdroot,get_param(gcb,'upperLimit'));
      |   if (upperLimit<=lowerLimit)
      |     warning('UpperLimit should be greater than LowerLimit.');
      |   end
      |   fltPropGain=pgain;
      |   fltIntegGain=igain*SampleTime*0.5;
      |   exparg=-SampleTime*filtCoef;
      |   expconst=exp(exparg);
      |   fltFiltCoef=expconst;
      |   fltDerivGain=dgain/SampleTime*(1 - expconst);
      |   fltUpperLimit=upperLimit;
      |   fltLowerLimit=lowerLimit;
      |   if isnan(fltPropGain)
      |     if ~strcmp(fltPropGain_bkup,'0')
      |       set_param(gcb,'fltPropGain','0');
      |     end
      |   else
      |     tmps=num2str(fltPropGain);
      |     if ~strcmp(fltPropGain_bkup,tmps)
      |       set_param(gcb,'fltPropGain',tmps);
      |     end
      |   end
      |   if isnan(fltIntegGain)
      |     if ~strcmp(fltIntegGain_bkup,'0')
      |       set_param(gcb,'fltIntegGain','0');
      |     end
      |   else
      |     tmps=num2str(fltIntegGain);
      |     if ~strcmp(fltIntegGain_bkup,tmps)
      |       set_param(gcb,'fltIntegGain',tmps);
      |     end
      |   end
      |   if isnan(fltDerivGain)
      |     if ~strcmp(fltDerivGain_bkup,'0')
      |       set_param(gcb,'fltDerivGain','0');
      |     end
      |   else
      |     tmps=num2str(fltDerivGain);
      |     if ~strcmp(fltDerivGain_bkup,tmps)
      |       set_param(gcb,'fltDerivGain',tmps);
      |     end
      |   end
      |   if isnan(fltFiltCoef)
      |     if ~strcmp(fltFiltCoef_bkup,'0')
      |       set_param(gcb,'fltFiltCoef','0');
      |     end
      |   else
      |     tmps=num2str(fltFiltCoef);
      |     if ~strcmp(fltFiltCoef_bkup,tmps)
      |       set_param(gcb,'fltFiltCoef',tmps);
      |     end
      |   end
      |   if isnan(fltLowerLimit)
      |     if ~strcmp(fltLowerLimit_bkup,'0')
      |       set_param(gcb,'fltLowerLimit','0');
      |     end
      |   else
      |     tmps=num2str(fltLowerLimit);
      |     if ~strcmp(fltLowerLimit_bkup,tmps)
      |       set_param(gcb,'fltLowerLimit',tmps);
      |     end
      |   end
      |   if isnan(fltUpperLimit)
      |     if ~strcmp(fltUpperLimit_bkup,'0')
      |       set_param(gcb,'fltUpperLimit','0');
      |     end
      |   else
      |     tmps=num2str(fltUpperLimit);
      |     if ~strcmp(fltUpperLimit_bkup,tmps)
      |       set_param(gcb,'fltUpperLimit',tmps);
      |     end
      |   end
      | end
      mask Callback dgain:
      | autoCalcEn=get_param(gcb,'autoCalcEn');
      | if strcmp(autoCalcEn,'on')
      |   SampleTime=Simulink.data.evalinGlobal(bdroot,get_param(gcb,'SampleTime'));
      |   if (SampleTime==-1)
      |     SampleTime=str2double(get_param(gcb,'SampleTime_1'));
      |   end
      |   fltPropGain_bkup=get_param(gcb,'fltPropGain');
      |   fltIntegGain_bkup=get_param(gcb,'fltIntegGain');
      |   fltDerivGain_bkup=get_param(gcb,'fltDerivGain');
      |   fltFiltCoef_bkup=get_param(gcb,'fltFiltCoef');
      |   fltLowerLimit_bkup=get_param(gcb,'fltLowerLimit');
      |   fltUpperLimit_bkup=get_param(gcb,'fltUpperLimit');
      |   pgain=Simulink.data.evalinGlobal(bdroot,get_param(gcb,'pgain'));
      |   igain=Simulink.data.evalinGlobal(bdroot,get_param(gcb,'igain'));
      |   dgain=Simulink.data.evalinGlobal(bdroot,get_param(gcb,'dgain'));
      |   filtCoef=Simulink.data.evalinGlobal(bdroot,get_param(gcb,'filtCoef'));
      |   lowerLimit=Simulink.data.evalinGlobal(bdroot,get_param(gcb,'lowerLimit'));
      |   upperLimit=Simulink.data.evalinGlobal(bdroot,get_param(gcb,'upperLimit'));
      |   if (upperLimit<=lowerLimit)
      |     warning('UpperLimit should be greater than LowerLimit.');
      |   end
      |   fltPropGain=pgain;
      |   fltIntegGain=igain*SampleTime*0.5;
      |   exparg=-SampleTime*filtCoef;
      |   expconst=exp(exparg);
      |   fltFiltCoef=expconst;
      |   fltDerivGain=dgain/SampleTime*(1 - expconst);
      |   fltUpperLimit=upperLimit;
      |   fltLowerLimit=lowerLimit;
      |   if isnan(fltPropGain)
      |     if ~strcmp(fltPropGain_bkup,'0')
      |       set_param(gcb,'fltPropGain','0');
      |     end
      |   else
      |     tmps=num2str(fltPropGain);
      |     if ~strcmp(fltPropGain_bkup,tmps)
      |       set_param(gcb,'fltPropGain',tmps);
      |     end
      |   end
      |   if isnan(fltIntegGain)
      |     if ~strcmp(fltIntegGain_bkup,'0')
      |       set_param(gcb,'fltIntegGain','0');
      |     end
      |   else
      |     tmps=num2str(fltIntegGain);
      |     if ~strcmp(fltIntegGain_bkup,tmps)
      |       set_param(gcb,'fltIntegGain',tmps);
      |     end
      |   end
      |   if isnan(fltDerivGain)
      |     if ~strcmp(fltDerivGain_bkup,'0')
      |       set_param(gcb,'fltDerivGain','0');
      |     end
      |   else
      |     tmps=num2str(fltDerivGain);
      |     if ~strcmp(fltDerivGain_bkup,tmps)
      |       set_param(gcb,'fltDerivGain',tmps);
      |     end
      |   end
      |   if isnan(fltFiltCoef)
      |     if ~strcmp(fltFiltCoef_bkup,'0')
      |       set_param(gcb,'fltFiltCoef','0');
      |     end
      |   else
      |     tmps=num2str(fltFiltCoef);
      |     if ~strcmp(fltFiltCoef_bkup,tmps)
      |       set_param(gcb,'fltFiltCoef',tmps);
      |     end
      |   end
      |   if isnan(fltLowerLimit)
      |     if ~strcmp(fltLowerLimit_bkup,'0')
      |       set_param(gcb,'fltLowerLimit','0');
      |     end
      |   else
      |     tmps=num2str(fltLowerLimit);
      |     if ~strcmp(fltLowerLimit_bkup,tmps)
      |       set_param(gcb,'fltLowerLimit',tmps);
      |     end
      |   end
      |   if isnan(fltUpperLimit)
      |     if ~strcmp(fltUpperLimit_bkup,'0')
      |       set_param(gcb,'fltUpperLimit','0');
      |     end
      |   else
      |     tmps=num2str(fltUpperLimit);
      |     if ~strcmp(fltUpperLimit_bkup,tmps)
      |       set_param(gcb,'fltUpperLimit',tmps);
      |     end
      |   end
      | end
      mask Callback filtCoef:
      | autoCalcEn=get_param(gcb,'autoCalcEn');
      | if strcmp(autoCalcEn,'on')
      |   SampleTime=Simulink.data.evalinGlobal(bdroot,get_param(gcb,'SampleTime'));
      |   if (SampleTime==-1)
      |     SampleTime=str2double(get_param(gcb,'SampleTime_1'));
      |   end
      |   fltPropGain_bkup=get_param(gcb,'fltPropGain');
      |   fltIntegGain_bkup=get_param(gcb,'fltIntegGain');
      |   fltDerivGain_bkup=get_param(gcb,'fltDerivGain');
      |   fltFiltCoef_bkup=get_param(gcb,'fltFiltCoef');
      |   fltLowerLimit_bkup=get_param(gcb,'fltLowerLimit');
      |   fltUpperLimit_bkup=get_param(gcb,'fltUpperLimit');
      |   pgain=Simulink.data.evalinGlobal(bdroot,get_param(gcb,'pgain'));
      |   igain=Simulink.data.evalinGlobal(bdroot,get_param(gcb,'igain'));
      |   dgain=Simulink.data.evalinGlobal(bdroot,get_param(gcb,'dgain'));
      |   filtCoef=Simulink.data.evalinGlobal(bdroot,get_param(gcb,'filtCoef'));
      |   lowerLimit=Simulink.data.evalinGlobal(bdroot,get_param(gcb,'lowerLimit'));
      |   upperLimit=Simulink.data.evalinGlobal(bdroot,get_param(gcb,'upperLimit'));
      |   if (upperLimit<=lowerLimit)
      |     warning('UpperLimit should be greater than LowerLimit.');
      |   end
      |   fltPropGain=pgain;
      |   fltIntegGain=igain*SampleTime*0.5;
      |   exparg=-SampleTime*filtCoef;
      |   expconst=exp(exparg);
      |   fltFiltCoef=expconst;
      |   fltDerivGain=dgain/SampleTime*(1 - expconst);
      |   fltUpperLimit=upperLimit;
      |   fltLowerLimit=lowerLimit;
      |   if isnan(fltPropGain)
      |     if ~strcmp(fltPropGain_bkup,'0')
      |       set_param(gcb,'fltPropGain','0');
      |     end
      |   else
      |     tmps=num2str(fltPropGain);
      |     if ~strcmp(fltPropGain_bkup,tmps)
      |       set_param(gcb,'fltPropGain',tmps);
      |     end
      |   end
      |   if isnan(fltIntegGain)
      |     if ~strcmp(fltIntegGain_bkup,'0')
      |       set_param(gcb,'fltIntegGain','0');
      |     end
      |   else
      |     tmps=num2str(fltIntegGain);
      |     if ~strcmp(fltIntegGain_bkup,tmps)
      |       set_param(gcb,'fltIntegGain',tmps);
      |     end
      |   end
      |   if isnan(fltDerivGain)
      |     if ~strcmp(fltDerivGain_bkup,'0')
      |       set_param(gcb,'fltDerivGain','0');
      |     end
      |   else
      |     tmps=num2str(fltDerivGain);
      |     if ~strcmp(fltDerivGain_bkup,tmps)
      |       set_param(gcb,'fltDerivGain',tmps);
      |     end
      |   end
      |   if isnan(fltFiltCoef)
      |     if ~strcmp(fltFiltCoef_bkup,'0')
      |       set_param(gcb,'fltFiltCoef','0');
      |     end
      |   else
      |     tmps=num2str(fltFiltCoef);
      |     if ~strcmp(fltFiltCoef_bkup,tmps)
      |       set_param(gcb,'fltFiltCoef',tmps);
      |     end
      |   end
      |   if isnan(fltLowerLimit)
      |     if ~strcmp(fltLowerLimit_bkup,'0')
      |       set_param(gcb,'fltLowerLimit','0');
      |     end
      |   else
      |     tmps=num2str(fltLowerLimit);
      |     if ~strcmp(fltLowerLimit_bkup,tmps)
      |       set_param(gcb,'fltLowerLimit',tmps);
      |     end
      |   end
      |   if isnan(fltUpperLimit)
      |     if ~strcmp(fltUpperLimit_bkup,'0')
      |       set_param(gcb,'fltUpperLimit','0');
      |     end
      |   else
      |     tmps=num2str(fltUpperLimit);
      |     if ~strcmp(fltUpperLimit_bkup,tmps)
      |       set_param(gcb,'fltUpperLimit',tmps);
      |     end
      |   end
      | end
      mask Callback lowerLimit:
      | autoCalcEn=get_param(gcb,'autoCalcEn');
      | if strcmp(autoCalcEn,'on')
      |   SampleTime=Simulink.data.evalinGlobal(bdroot,get_param(gcb,'SampleTime'));
      |   if (SampleTime==-1)
      |     SampleTime=str2double(get_param(gcb,'SampleTime_1'));
      |   end
      |   fltPropGain_bkup=get_param(gcb,'fltPropGain');
      |   fltIntegGain_bkup=get_param(gcb,'fltIntegGain');
      |   fltDerivGain_bkup=get_param(gcb,'fltDerivGain');
      |   fltFiltCoef_bkup=get_param(gcb,'fltFiltCoef');
      |   fltLowerLimit_bkup=get_param(gcb,'fltLowerLimit');
      |   fltUpperLimit_bkup=get_param(gcb,'fltUpperLimit');
      |   pgain=Simulink.data.evalinGlobal(bdroot,get_param(gcb,'pgain'));
      |   igain=Simulink.data.evalinGlobal(bdroot,get_param(gcb,'igain'));
      |   dgain=Simulink.data.evalinGlobal(bdroot,get_param(gcb,'dgain'));
      |   filtCoef=Simulink.data.evalinGlobal(bdroot,get_param(gcb,'filtCoef'));
      |   lowerLimit=Simulink.data.evalinGlobal(bdroot,get_param(gcb,'lowerLimit'));
      |   upperLimit=Simulink.data.evalinGlobal(bdroot,get_param(gcb,'upperLimit'));
      |   if (upperLimit<=lowerLimit)
      |     warning('UpperLimit should be greater than LowerLimit.');
      |   end
      |   fltPropGain=pgain;
      |   fltIntegGain=igain*SampleTime*0.5;
      |   exparg=-SampleTime*filtCoef;
      |   expconst=exp(exparg);
      |   fltFiltCoef=expconst;
      |   fltDerivGain=dgain/SampleTime*(1 - expconst);
      |   fltUpperLimit=upperLimit;
      |   fltLowerLimit=lowerLimit;
      |   if isnan(fltPropGain)
      |     if ~strcmp(fltPropGain_bkup,'0')
      |       set_param(gcb,'fltPropGain','0');
      |     end
      |   else
      |     tmps=num2str(fltPropGain);
      |     if ~strcmp(fltPropGain_bkup,tmps)
      |       set_param(gcb,'fltPropGain',tmps);
      |     end
      |   end
      |   if isnan(fltIntegGain)
      |     if ~strcmp(fltIntegGain_bkup,'0')
      |       set_param(gcb,'fltIntegGain','0');
      |     end
      |   else
      |     tmps=num2str(fltIntegGain);
      |     if ~strcmp(fltIntegGain_bkup,tmps)
      |       set_param(gcb,'fltIntegGain',tmps);
      |     end
      |   end
      |   if isnan(fltDerivGain)
      |     if ~strcmp(fltDerivGain_bkup,'0')
      |       set_param(gcb,'fltDerivGain','0');
      |     end
      |   else
      |     tmps=num2str(fltDerivGain);
      |     if ~strcmp(fltDerivGain_bkup,tmps)
      |       set_param(gcb,'fltDerivGain',tmps);
      |     end
      |   end
      |   if isnan(fltFiltCoef)
      |     if ~strcmp(fltFiltCoef_bkup,'0')
      |       set_param(gcb,'fltFiltCoef','0');
      |     end
      |   else
      |     tmps=num2str(fltFiltCoef);
      |     if ~strcmp(fltFiltCoef_bkup,tmps)
      |       set_param(gcb,'fltFiltCoef',tmps);
      |     end
      |   end
      |   if isnan(fltLowerLimit)
      |     if ~strcmp(fltLowerLimit_bkup,'0')
      |       set_param(gcb,'fltLowerLimit','0');
      |     end
      |   else
      |     tmps=num2str(fltLowerLimit);
      |     if ~strcmp(fltLowerLimit_bkup,tmps)
      |       set_param(gcb,'fltLowerLimit',tmps);
      |     end
      |   end
      |   if isnan(fltUpperLimit)
      |     if ~strcmp(fltUpperLimit_bkup,'0')
      |       set_param(gcb,'fltUpperLimit','0');
      |     end
      |   else
      |     tmps=num2str(fltUpperLimit);
      |     if ~strcmp(fltUpperLimit_bkup,tmps)
      |       set_param(gcb,'fltUpperLimit',tmps);
      |     end
      |   end
      | end
      mask Callback upperLimit:
      | autoCalcEn=get_param(gcb,'autoCalcEn');
      | if strcmp(autoCalcEn,'on')
      |   SampleTime=Simulink.data.evalinGlobal(bdroot,get_param(gcb,'SampleTime'));
      |   if (SampleTime==-1)
      |     SampleTime=str2double(get_param(gcb,'SampleTime_1'));
      |   end
      |   fltPropGain_bkup=get_param(gcb,'fltPropGain');
      |   fltIntegGain_bkup=get_param(gcb,'fltIntegGain');
      |   fltDerivGain_bkup=get_param(gcb,'fltDerivGain');
      |   fltFiltCoef_bkup=get_param(gcb,'fltFiltCoef');
      |   fltLowerLimit_bkup=get_param(gcb,'fltLowerLimit');
      |   fltUpperLimit_bkup=get_param(gcb,'fltUpperLimit');
      |   pgain=Simulink.data.evalinGlobal(bdroot,get_param(gcb,'pgain'));
      |   igain=Simulink.data.evalinGlobal(bdroot,get_param(gcb,'igain'));
      |   dgain=Simulink.data.evalinGlobal(bdroot,get_param(gcb,'dgain'));
      |   filtCoef=Simulink.data.evalinGlobal(bdroot,get_param(gcb,'filtCoef'));
      |   lowerLimit=Simulink.data.evalinGlobal(bdroot,get_param(gcb,'lowerLimit'));
      |   upperLimit=Simulink.data.evalinGlobal(bdroot,get_param(gcb,'upperLimit'));
      |   if (upperLimit<=lowerLimit)
      |     warning('UpperLimit should be greater than LowerLimit.');
      |   end
      |   fltPropGain=pgain;
      |   fltIntegGain=igain*SampleTime*0.5;
      |   exparg=-SampleTime*filtCoef;
      |   expconst=exp(exparg);
      |   fltFiltCoef=expconst;
      |   fltDerivGain=dgain/SampleTime*(1 - expconst);
      |   fltUpperLimit=upperLimit;
      |   fltLowerLimit=lowerLimit;
      |   if isnan(fltPropGain)
      |     if ~strcmp(fltPropGain_bkup,'0')
      |       set_param(gcb,'fltPropGain','0');
      |     end
      |   else
      |     tmps=num2str(fltPropGain);
      |     if ~strcmp(fltPropGain_bkup,tmps)
      |       set_param(gcb,'fltPropGain',tmps);
      |     end
      |   end
      |   if isnan(fltIntegGain)
      |     if ~strcmp(fltIntegGain_bkup,'0')
      |       set_param(gcb,'fltIntegGain','0');
      |     end
      |   else
      |     tmps=num2str(fltIntegGain);
      |     if ~strcmp(fltIntegGain_bkup,tmps)
      |       set_param(gcb,'fltIntegGain',tmps);
      |     end
      |   end
      |   if isnan(fltDerivGain)
      |     if ~strcmp(fltDerivGain_bkup,'0')
      |       set_param(gcb,'fltDerivGain','0');
      |     end
      |   else
      |     tmps=num2str(fltDerivGain);
      |     if ~strcmp(fltDerivGain_bkup,tmps)
      |       set_param(gcb,'fltDerivGain',tmps);
      |     end
      |   end
      |   if isnan(fltFiltCoef)
      |     if ~strcmp(fltFiltCoef_bkup,'0')
      |       set_param(gcb,'fltFiltCoef','0');
      |     end
      |   else
      |     tmps=num2str(fltFiltCoef);
      |     if ~strcmp(fltFiltCoef_bkup,tmps)
      |       set_param(gcb,'fltFiltCoef',tmps);
      |     end
      |   end
      |   if isnan(fltLowerLimit)
      |     if ~strcmp(fltLowerLimit_bkup,'0')
      |       set_param(gcb,'fltLowerLimit','0');
      |     end
      |   else
      |     tmps=num2str(fltLowerLimit);
      |     if ~strcmp(fltLowerLimit_bkup,tmps)
      |       set_param(gcb,'fltLowerLimit',tmps);
      |     end
      |   end
      |   if isnan(fltUpperLimit)
      |     if ~strcmp(fltUpperLimit_bkup,'0')
      |       set_param(gcb,'fltUpperLimit','0');
      |     end
      |   else
      |     tmps=num2str(fltUpperLimit);
      |     if ~strcmp(fltUpperLimit_bkup,tmps)
      |       set_param(gcb,'fltUpperLimit',tmps);
      |     end
      |   end
      | end
      mask Callback autoCalcEn:
      | maskStr=get_param(gcb,'showStates');
      | if strcmp(maskStr,'Hide (faster execution)')
      |   p=Simulink.Mask.get(gcb);
      |   autoCalcEn=get_param(gcb,'autoCalcEn');
      |   hintText=p.getDialogControl('timeHint');
      |   if strcmp(autoCalcEn,'on')
      |     param=p.getParameter('upperLimit');
      |     if strcmp(param.Enabled,'off')
      |       SampleTime=Simulink.data.evalinGlobal(bdroot,get_param(gcb,'SampleTime'));
      |       if SampleTime==-1
      |         SampleTime=str2double(get_param(gcb,'SampleTime_1'));
      |         if isnan(SampleTime)
      |           hintText.Prompt=['Note: Implementation parameters cannot be calculated yet because the block''s inherited sample time is unknown. Simulink will update the sample time when you run the simulation.'];
      |         else
      |           hintText.Prompt=['Caution: Implementation parameters depend on inherited sample time. Make sure that the sample time of the block''s inputs corresponds to the sampling period in the target application.'];
      |         end
      |       else
      |         hintText.Prompt='Caution: Implementation parameters depend on the sample time. Make sure that the simulation time step corresponds to the sampling period in the target application.';
      |       end
      |       p=Simulink.Mask.get(gcb);
      |       param=p.getParameter('pgain');
      |       param.set('Enabled','on');
      |       param=p.getParameter('igain');
      |       param.set('Enabled','on');
      |       param=p.getParameter('dgain');
      |       param.set('Enabled','on');
      |       param=p.getParameter('filtCoef');
      |       param.set('Enabled','on');
      |       param=p.getParameter('lowerLimit');
      |       param.set('Enabled','on');
      |       param=p.getParameter('upperLimit');
      |       param.set('Enabled','on');
      |     else
      |       SampleTime=Simulink.data.evalinGlobal(bdroot,get_param(gcb,'SampleTime'));
      |       if SampleTime==-1
      |         SampleTime=str2double(get_param(gcb,'SampleTime_1'));
      |       end
      |     end
      |     fltPropGain_bkup=get_param(gcb,'fltPropGain');
      |     fltIntegGain_bkup=get_param(gcb,'fltIntegGain');
      |     fltDerivGain_bkup=get_param(gcb,'fltDerivGain');
      |     fltFiltCoef_bkup=get_param(gcb,'fltFiltCoef');
      |     fltLowerLimit_bkup=get_param(gcb,'fltLowerLimit');
      |     fltUpperLimit_bkup=get_param(gcb,'fltUpperLimit');
      |     pgain=Simulink.data.evalinGlobal(bdroot,get_param(gcb,'pgain'));
      |     igain=Simulink.data.evalinGlobal(bdroot,get_param(gcb,'igain'));
      |     dgain=Simulink.data.evalinGlobal(bdroot,get_param(gcb,'dgain'));
      |     filtCoef=Simulink.data.evalinGlobal(bdroot,get_param(gcb,'filtCoef'));
      |     lowerLimit=Simulink.data.evalinGlobal(bdroot,get_param(gcb,'lowerLimit'));
      |     upperLimit=Simulink.data.evalinGlobal(bdroot,get_param(gcb,'upperLimit'));
      |     if (upperLimit<=lowerLimit)
      |       warning('UpperLimit should be greater than LowerLimit.');
      |     end
      |     fltPropGain=pgain;
      |     fltIntegGain=igain*SampleTime*0.5;
      |     exparg=-SampleTime*filtCoef;
      |     expconst=exp(exparg);
      |     fltFiltCoef=expconst;
      |     fltDerivGain=dgain/SampleTime*(1 - expconst);
      |     fltUpperLimit=upperLimit;
      |     fltLowerLimit=lowerLimit;
      |     if isnan(fltPropGain)
      |       if ~strcmp(fltPropGain_bkup,'0')
      |         set_param(gcb,'fltPropGain','0');
      |       end
      |     else
      |       tmps=num2str(fltPropGain);
      |       if ~strcmp(fltPropGain_bkup,tmps)
      |         set_param(gcb,'fltPropGain',tmps);
      |       end
      |     end
      |     if isnan(fltIntegGain)
      |       if ~strcmp(fltIntegGain_bkup,'0')
      |         set_param(gcb,'fltIntegGain','0');
      |       end
      |     else
      |       tmps=num2str(fltIntegGain);
      |       if ~strcmp(fltIntegGain_bkup,tmps)
      |         set_param(gcb,'fltIntegGain',tmps);
      |       end
      |     end
      |     if isnan(fltDerivGain)
      |       if ~strcmp(fltDerivGain_bkup,'0')
      |         set_param(gcb,'fltDerivGain','0');
      |       end
      |     else
      |       tmps=num2str(fltDerivGain);
      |       if ~strcmp(fltDerivGain_bkup,tmps)
      |         set_param(gcb,'fltDerivGain',tmps);
      |       end
      |     end
      |     if isnan(fltFiltCoef)
      |       if ~strcmp(fltFiltCoef_bkup,'0')
      |         set_param(gcb,'fltFiltCoef','0');
      |       end
      |     else
      |       tmps=num2str(fltFiltCoef);
      |       if ~strcmp(fltFiltCoef_bkup,tmps)
      |         set_param(gcb,'fltFiltCoef',tmps);
      |       end
      |     end
      |     if isnan(fltLowerLimit)
      |       if ~strcmp(fltLowerLimit_bkup,'0')
      |         set_param(gcb,'fltLowerLimit','0');
      |       end
      |     else
      |       tmps=num2str(fltLowerLimit);
      |       if ~strcmp(fltLowerLimit_bkup,tmps)
      |         set_param(gcb,'fltLowerLimit',tmps);
      |       end
      |     end
      |     if isnan(fltUpperLimit)
      |       if ~strcmp(fltUpperLimit_bkup,'0')
      |         set_param(gcb,'fltUpperLimit','0');
      |       end
      |     else
      |       tmps=num2str(fltUpperLimit);
      |       if ~strcmp(fltUpperLimit_bkup,tmps)
      |         set_param(gcb,'fltUpperLimit',tmps);
      |       end
      |     end
      |   else
      |     param=p.getParameter('upperLimit');
      |     if strcmp(param.Enabled,'on')
      |       hintText.Prompt='Caution: Implementation parameters are fixed.';
      |       p=Simulink.Mask.get(gcb);
      |       param=p.getParameter('pgain');
      |       param.set('Enabled','off');
      |       param=p.getParameter('igain');
      |       param.set('Enabled','off');
      |       param=p.getParameter('dgain');
      |       param.set('Enabled','off');
      |       param=p.getParameter('filtCoef');
      |       param.set('Enabled','off');
      |       param=p.getParameter('lowerLimit');
      |       param.set('Enabled','off');
      |       param=p.getParameter('upperLimit');
      |       param.set('Enabled','off');
      |     end
      |   end
      | end
      mask DialogControl CompBut Prompt: Recalculate sample times
      mask DialogControl CompBut Tooltip: Simulink updates the sample times of all blocks when the simulation is run. This button will update the sample times now.
      mask DialogControl CompBut Callback:
      | btn=questdlg('This will apply all changes in all open dialog boxes and update the schematic. Do you want to proceed?','Apply all changes','Continue','Cancel','Continue');
      | if strcmp(btn,'Continue')
      |   dlgs=DAStudio.ToolRoot.getOpenDialogs;
      |   for i=1:length(dlgs)
      |     dlgs(i).apply;
      |   end
      |   try
      |     SampleTime_1=str2double(get_param(gcb,'SampleTime_1'));
      |     ts=Simulink.Block.getSampleTimes(gcb);
      |     ts=ts(1).Value(1);
      |     if (SampleTime_1 ~= ts)
      |       SampleTime_1=ts;
      |       set_param(gcb,'SampleTime_1',num2str(ts));
      |       autoCalcEn=get_param(gcb,'autoCalcEn');
      |       if strcmp(autoCalcEn,'on')
      |         SampleTime=Simulink.data.evalinGlobal(bdroot,get_param(gcb,'SampleTime'));
      |         p=Simulink.Mask.get(gcb);
      |         hintText=p.getDialogControl('timeHint');
      |         if SampleTime==-1
      |           SampleTime=SampleTime_1;
      |           hintText.Prompt='Caution: Implementation parameters depend on inherited sample time. Make sure that the sample time of the block''s inputs corresponds to the sampling period in the target application.';
      |         else
      |           hintText.Prompt='Caution: Implementation parameters depend on the sample time. Make sure that the simulation time step corresponds to the sampling period in the target application.';
      |         end
      |         fltPropGain_bkup=get_param(gcb,'fltPropGain');
      |         fltIntegGain_bkup=get_param(gcb,'fltIntegGain');
      |         fltDerivGain_bkup=get_param(gcb,'fltDerivGain');
      |         fltFiltCoef_bkup=get_param(gcb,'fltFiltCoef');
      |         fltLowerLimit_bkup=get_param(gcb,'fltLowerLimit');
      |         fltUpperLimit_bkup=get_param(gcb,'fltUpperLimit');
      |         pgain=Simulink.data.evalinGlobal(bdroot,get_param(gcb,'pgain'));
      |         igain=Simulink.data.evalinGlobal(bdroot,get_param(gcb,'igain'));
      |         dgain=Simulink.data.evalinGlobal(bdroot,get_param(gcb,'dgain'));
      |         filtCoef=Simulink.data.evalinGlobal(bdroot,get_param(gcb,'filtCoef'));
      |         lowerLimit=Simulink.data.evalinGlobal(bdroot,get_param(gcb,'lowerLimit'));
      |         upperLimit=Simulink.data.evalinGlobal(bdroot,get_param(gcb,'upperLimit'));
      |         if (upperLimit<=lowerLimit)
      |           warning('UpperLimit should be greater than LowerLimit.');
      |         end
      |         fltPropGain=pgain;
      |         fltIntegGain=igain*SampleTime*0.5;
      |         exparg=-SampleTime*filtCoef;
      |         expconst=exp(exparg);
      |         fltFiltCoef=expconst;
      |         fltDerivGain=dgain/SampleTime*(1 - expconst);
      |         fltUpperLimit=upperLimit;
      |         fltLowerLimit=lowerLimit;
      |         if isnan(fltPropGain)
      |           if ~strcmp(fltPropGain_bkup,'0')
      |             set_param(gcb,'fltPropGain','0');
      |           end
      |         else
      |           tmps=num2str(fltPropGain);
      |           if ~strcmp(fltPropGain_bkup,tmps)
      |             set_param(gcb,'fltPropGain',tmps);
      |           end
      |         end
      |         if isnan(fltIntegGain)
      |           if ~strcmp(fltIntegGain_bkup,'0')
      |             set_param(gcb,'fltIntegGain','0');
      |           end
      |         else
      |           tmps=num2str(fltIntegGain);
      |           if ~strcmp(fltIntegGain_bkup,tmps)
      |             set_param(gcb,'fltIntegGain',tmps);
      |           end
      |         end
      |         if isnan(fltDerivGain)
      |           if ~strcmp(fltDerivGain_bkup,'0')
      |             set_param(gcb,'fltDerivGain','0');
      |           end
      |         else
      |           tmps=num2str(fltDerivGain);
      |           if ~strcmp(fltDerivGain_bkup,tmps)
      |             set_param(gcb,'fltDerivGain',tmps);
      |           end
      |         end
      |         if isnan(fltFiltCoef)
      |           if ~strcmp(fltFiltCoef_bkup,'0')
      |             set_param(gcb,'fltFiltCoef','0');
      |           end
      |         else
      |           tmps=num2str(fltFiltCoef);
      |           if ~strcmp(fltFiltCoef_bkup,tmps)
      |             set_param(gcb,'fltFiltCoef',tmps);
      |           end
      |         end
      |         if isnan(fltLowerLimit)
      |           if ~strcmp(fltLowerLimit_bkup,'0')
      |             set_param(gcb,'fltLowerLimit','0');
      |           end
      |         else
      |           tmps=num2str(fltLowerLimit);
      |           if ~strcmp(fltLowerLimit_bkup,tmps)
      |             set_param(gcb,'fltLowerLimit',tmps);
      |           end
      |         end
      |         if isnan(fltUpperLimit)
      |           if ~strcmp(fltUpperLimit_bkup,'0')
      |             set_param(gcb,'fltUpperLimit','0');
      |           end
      |         else
      |           tmps=num2str(fltUpperLimit);
      |           if ~strcmp(fltUpperLimit_bkup,tmps)
      |             set_param(gcb,'fltUpperLimit',tmps);
      |           end
      |         end
      |       end
      |     end
      |   catch
      |    warning(['Sample time cannot be calculated for the block ' gcb])
      |   end
      | end
      mask DialogControl timeHint Prompt: Note: Implementation parameters cannot be calculated yet because the block's inherited sample time is unknown. Simulink will update the sample time when you run the simulation.
      mask Display:
      | color('black');
      | pos = get_param(gcb, 'Position');
      | width = pos(3) - pos(1);
      | height = pos(4) - pos(2);
      | tX=width/2;
      | tY=height - 25;
      | color('black');
      | text(tX,tY, 'GFLIB_ControllerPIDpAW_FLT', 'horizontalAlignment', 'center');
      | if showStates == 2
      |   color('red');
      |   text(tX,tY - 20, ['debugging mode' char(13) char(10) '(limited performance)'], 'horizontalAlignment', 'center');
      | end
  GFLIB_ControllerPIpAW_FLT : Subsystem  StartFcn=|  TreatAsAtomicUnit=on  mask(GFLIB_ControllerPIpAW_FLT){showStates=Hide (faster execution), resetStatesEnable=Pre-set according to the first set of inputs after reset, SampleTime=-1, pgain=5, igain=0.5, lowerLimit=-10, upperLimit=10, autoCalcEn=on, fltPropGain=0, fltIntegGain=0, fltLowerLimit=0, fltUpperLimit=0, SampleTime_1=NaN}
      | ts=get_param(gcb,'CompiledSampleTime');
      | if iscell(ts)
      |   ts=ts{1};
      |   if iscell(ts)
      |     ts=ts{1};
      |   end
      | end
      | ts=ts(1);
      | set_param(gcb,'SampleTime_1',num2str(ts));
      | p=Simulink.Mask.get(gcb);
      | hintText=p.getDialogControl('timeHint');
      | SampleTime=Simulink.data.evalinGlobal(bdroot,get_param(gcb,'SampleTime'));
      | p=Simulink.Mask.get(gcb);
      | autoCalcEn=get_param(gcb,'autoCalcEn');
      | if strcmp(autoCalcEn,'on')
      |   if SampleTime==-1
      |     hintText.Prompt='Caution: Implementation parameters depend on inherited sample time. Make sure that the sample time of the block''s inputs corresponds to the sampling period in the target application.';
      |   else
      |     hintText.Prompt='Caution: Implementation parameters depend on the sample time. Make sure that the simulation time step corresponds to the sampling period in the target application.';
      |   end
      |   SampleTime=ts;
      |   fltPropGain_bkup=get_param(gcb,'fltPropGain');
      |   fltIntegGain_bkup=get_param(gcb,'fltIntegGain');
      |   fltLowerLimit_bkup=get_param(gcb,'fltLowerLimit');
      |   fltUpperLimit_bkup=get_param(gcb,'fltUpperLimit');
      |   pgain=Simulink.data.evalinGlobal(bdroot,get_param(gcb,'pgain'));
      |   igain=Simulink.data.evalinGlobal(bdroot,get_param(gcb,'igain'));
      |   lowerLimit=Simulink.data.evalinGlobal(bdroot,get_param(gcb,'lowerLimit'));
      |   upperLimit=Simulink.data.evalinGlobal(bdroot,get_param(gcb,'upperLimit'));
      |   if (upperLimit<=lowerLimit)
      |     warning('UpperLimit should be greater than LowerLimit.');
      |   end
      |   fltPropGain=pgain;
      |   fltIntegGain=igain*SampleTime*0.5;
      |   fltUpperLimit=upperLimit;
      |   fltLowerLimit=lowerLimit;
      |   if isnan(fltPropGain)
      |     if ~strcmp(fltPropGain_bkup,'0')
      |       set_param(gcb,'fltPropGain','0');
      |     end
      |   else
      |     tmps=num2str(fltPropGain);
      |     if ~strcmp(fltPropGain_bkup,tmps)
      |       set_param(gcb,'fltPropGain',tmps);
      |     end
      |   end
      |   if isnan(fltIntegGain)
      |     if ~strcmp(fltIntegGain_bkup,'0')
      |       set_param(gcb,'fltIntegGain','0');
      |     end
      |   else
      |     tmps=num2str(fltIntegGain);
      |     if ~strcmp(fltIntegGain_bkup,tmps)
      |       set_param(gcb,'fltIntegGain',tmps);
      |     end
      |   end
      |   if isnan(fltLowerLimit)
      |     if ~strcmp(fltLowerLimit_bkup,'0')
      |       set_param(gcb,'fltLowerLimit','0');
      |     end
      |   else
      |     tmps=num2str(fltLowerLimit);
      |     if ~strcmp(fltLowerLimit_bkup,tmps)
      |       set_param(gcb,'fltLowerLimit',tmps);
      |     end
      |   end
      |   if isnan(fltUpperLimit)
      |     if ~strcmp(fltUpperLimit_bkup,'0')
      |       set_param(gcb,'fltUpperLimit','0');
      |     end
      |   else
      |     tmps=num2str(fltUpperLimit);
      |     if ~strcmp(fltUpperLimit_bkup,tmps)
      |       set_param(gcb,'fltUpperLimit',tmps);
      |     end
      |   end
      | end
      mask prompts: showStates "Show internal states:"; resetStatesEnable "Internal state after reset:"; SampleTime "Sample time (-1 for inherited):"; pgain "Proportional gain (P):"; igain "Integral gain (I):"; lowerLimit "Controller lower limit:"; upperLimit "Controller upper limit:"; autoCalcEn "Calculate implementation parameters from physical parameters"; fltPropGain "fltPropGain (Proportional gain):"; fltIntegGain "fltIntegGain (Integral gain):"; fltLowerLimit "fltLowerLimit (Lower Limit of the controller):"; fltUpperLimit "fltUpperLimit (Upper Limit of the controller):"; SampleTime_1 "Discrete sample time:"
      mask help: Parallel form discrete-time PI controller with anti-windup in single precision floating-point implementation. This block supports re-initialization of the internal state during simulation. If the block is reset, the controller's output will be aligned with the input fltControllerPIpAWOut_preset. Refer to the AMMCLIB User's Guide for further details.
      mask init:
      | ddName = get_param(bdroot,'DataDictionary');
      | if length(ddName)==0
      |   set_param(bdroot,'DataDictionary','ammclib_types.sldd');
      | else
      |   dd = Simulink.data.dictionary.open(ddName);
      |   data = getSection(dd,'Design Data');
      |   if ~exist(data,'SWLIBS_2Syst_F16')
      |     addDataSource(dd,'ammclib_types.sldd');
      |     saveChanges(dd);
      |   end
      | end
      | 
      | if showStates == 1
      |   % hidden state variables
      |   if strcmp(get_param([gcb '/fltPropGain'], 'BlockType'), 'Inport')
      |     posblk = get_param(gcb, 'Position');
      | 
      |     pos = get_param([gcb, '/fltPropGain'], 'Position');
      |     orient = get_param([gcb, '/fltPropGain'], 'Orientation');
      |     delete_block([gcb, '/fltPropGain']);
      |     add_block('built-in/Ground', [gcb, '/fltPropGain'], 'Position', pos, 'Orientation', orient);
      | 
      |     pos = get_param([gcb, '/fltIntegGain'], 'Position');
      |     orient = get_param([gcb, '/fltIntegGain'], 'Orientation');
      |     delete_block([gcb, '/fltIntegGain']);
      |     add_block('built-in/Ground', [gcb, '/fltIntegGain'], 'Position', pos, 'Orientation', orient);
      | 
      |     pos = get_param([gcb, '/fltLowerLimit'], 'Position');
      |     orient = get_param([gcb, '/fltLowerLimit'], 'Orientation');
      |     delete_block([gcb, '/fltLowerLimit']);
      |     add_block('built-in/Ground', [gcb, '/fltLowerLimit'], 'Position', pos, 'Orientation', orient);
      | 
      |     pos = get_param([gcb, '/fltUpperLimit'], 'Position');
      |     orient = get_param([gcb, '/fltUpperLimit'], 'Orientation');
      |     delete_block([gcb, '/fltUpperLimit']);
      |     add_block('built-in/Ground', [gcb, '/fltUpperLimit'], 'Position', pos, 'Orientation', orient);
      | 
      |     pos = get_param([gcb, '/fltIntegPartK_1'], 'Position');
      |     orient = get_param([gcb, '/fltIntegPartK_1'], 'Orientation');
      |     delete_block([gcb, '/fltIntegPartK_1']);
      |     add_block('built-in/Ground', [gcb, '/fltIntegPartK_1'], 'Position', pos, 'Orientation', orient);
      | 
      |     pos = get_param([gcb, '/fltInK_1'], 'Position');
      |     orient = get_param([gcb, '/fltInK_1'], 'Orientation');
      |     delete_block([gcb, '/fltInK_1']);
      |     add_block('built-in/Ground', [gcb, '/fltInK_1'], 'Position', pos, 'Orientation', orient);
      | 
      | 
      |     pmask=Simulink.Mask.get(gcb);
      |     pctrl=pmask.getParameter('SampleTime');
      |     pctrl.set('TypeOptions',{'fltInErr/SampleTime','fltControllerPIpAWOut_preset/SampleTime'});
      | 
      |     pos = get_param([gcb '/fltIntegPartK_1_Out'], 'Position');
      |     orient = get_param([gcb '/fltIntegPartK_1_Out'], 'Orientation');
      |     delete_block([gcb '/fltIntegPartK_1_Out']);
      |     add_block('built-in/Terminator', [gcb '/fltIntegPartK_1_Out'], 'Position', pos, 'Orientation', orient);
      | 
      |     pos = get_param([gcb '/fltInK_1_Out'], 'Position');
      |     orient = get_param([gcb '/fltInK_1_Out'], 'Orientation');
      |     delete_block([gcb '/fltInK_1_Out']);
      |     add_block('built-in/Terminator', [gcb '/fltInK_1_Out'], 'Position', pos, 'Orientation', orient);
      | 
      |     set_param([gcb '/fltInErr'], 'Port', '1');
      |     set_param([gcb '/fltControllerPIpAWOut_preset'], 'Port', '2');
      | 
      |     tmpOutCnt=0;
      |     tmpOutCnt=tmpOutCnt+1;
      |     set_param([gcb '/fltOut'], 'Port', num2str(tmpOutCnt));
      |     tmpOutCnt=tmpOutCnt+1;
      |     set_param([gcb '/u16LimitFlag'], 'Port', num2str(tmpOutCnt));
      | 
      |     autoCalcEn=get_param(gcb,'autoCalcEn');
      |     if strcmp(autoCalcEn,'on')
      |       set_param(gcb,'MaskEnables',{'on','on','on','on','on','on','on','on','on','on','on','on','off'});
      |     else
      |       set_param(gcb,'MaskEnables',{'on','on','on','off','off','off','off','on','on','on','on','on','off'});
      |     end
      | 
      |     if (posblk(4) - posblk(2)) > 75
      |       height = 75;
      |       set_param(gcb,'Position',[posblk(1), posblk(2), posblk(3), posblk(2)+height])
      |     end
      |   end
      | else
      |   % shown state variables
      |   if strcmp(get_param([gcb '/fltPropGain'], 'BlockType'), 'Ground')
      |     posblk = get_param(gcb, 'Position');
      | 
      |     pos = get_param([gcb, '/fltPropGain'], 'Position');
      |     orient = get_param([gcb, '/fltPropGain'], 'Orientation');
      |     delete_block([gcb, '/fltPropGain']);
      |     add_block('built-in/Inport', [gcb, '/fltPropGain'], 'Position', pos, 'Orientation', orient, 'OutDataTypeStr', 'single');
      | 
      |     pos = get_param([gcb, '/fltIntegGain'], 'Position');
      |     orient = get_param([gcb, '/fltIntegGain'], 'Orientation');
      |     delete_block([gcb, '/fltIntegGain']);
      |     add_block('built-in/Inport', [gcb, '/fltIntegGain'], 'Position', pos, 'Orientation', orient, 'OutDataTypeStr', 'single');
      | 
      |     pos = get_param([gcb, '/fltLowerLimit'], 'Position');
      |     orient = get_param([gcb, '/fltLowerLimit'], 'Orientation');
      |     delete_block([gcb, '/fltLowerLimit']);
      |     add_block('built-in/Inport', [gcb, '/fltLowerLimit'], 'Position', pos, 'Orientation', orient, 'OutDataTypeStr', 'single');
      | 
      |     pos = get_param([gcb, '/fltUpperLimit'], 'Position');
      |     orient = get_param([gcb, '/fltUpperLimit'], 'Orientation');
      |     delete_block([gcb, '/fltUpperLimit']);
      |     add_block('built-in/Inport', [gcb, '/fltUpperLimit'], 'Position', pos, 'Orientation', orient, 'OutDataTypeStr', 'single');
      | 
      |     pos = get_param([gcb, '/fltIntegPartK_1'], 'Position');
      |     orient = get_param([gcb, '/fltIntegPartK_1'], 'Orientation');
      |     delete_block([gcb, '/fltIntegPartK_1']);
      |     add_block('built-in/Inport', [gcb, '/fltIntegPartK_1'], 'Position', pos, 'Orientation', orient, 'OutDataTypeStr', 'single');
      | 
      |     pos = get_param([gcb, '/fltInK_1'], 'Position');
      |     orient = get_param([gcb, '/fltInK_1'], 'Orientation');
      |     delete_block([gcb, '/fltInK_1']);
      |     add_block('built-in/Inport', [gcb, '/fltInK_1'], 'Position', pos, 'Orientation', orient, 'OutDataTypeStr', 'single');
      | 
      | 
      | 
      |     pos = get_param([gcb '/fltIntegPartK_1_Out'], 'Position');
      |     orient = get_param([gcb '/fltIntegPartK_1_Out'], 'Orientation');
      |     delete_block([gcb '/fltIntegPartK_1_Out']);
      |     add_block('built-in/Outport', [gcb '/fltIntegPartK_1_Out'], 'Position', pos, 'Orientation', orient);
      | 
      |     pos = get_param([gcb '/fltInK_1_Out'], 'Position');
      |     orient = get_param([gcb '/fltInK_1_Out'], 'Orientation');
      |     delete_block([gcb '/fltInK_1_Out']);
      |     add_block('built-in/Outport', [gcb '/fltInK_1_Out'], 'Position', pos, 'Orientation', orient);
      | 
      | 
      |     pmask=Simulink.Mask.get(gcb);
      |     pctrl=pmask.getParameter('SampleTime');
      |     pctrl.set('TypeOptions',{'fltInErr/SampleTime','fltControllerPIpAWOut_preset/SampleTime','fltPropGain/SampleTime','fltIntegGain/SampleTime','fltLowerLimit/SampleTime','fltUpperLimit/SampleTime','fltIntegPartK_1/SampleTime','fltInK_1/SampleTime'});
      | 
      |     set_param([gcb '/fltInErr'], 'Port', '1');
      |     set_param([gcb '/fltControllerPIpAWOut_preset'], 'Port', '2');
      |     set_param([gcb '/fltPropGain'], 'Port', '3');
      |     set_param([gcb '/fltIntegGain'], 'Port', '4');
      |     set_param([gcb '/fltLowerLimit'], 'Port', '5');
      |     set_param([gcb '/fltUpperLimit'], 'Port', '6');
      |     set_param([gcb '/fltIntegPartK_1'], 'Port', '7');
      |     set_param([gcb '/fltInK_1'], 'Port', '8');
      | 
      |     tmpOutCnt=0;
      |     tmpOutCnt=tmpOutCnt+1;
      |     set_param([gcb '/fltOut'], 'Port', num2str(tmpOutCnt));
      |     tmpOutCnt=tmpOutCnt+1;
      |     set_param([gcb '/u16LimitFlag'], 'Port', num2str(tmpOutCnt));
      |     tmpOutCnt=tmpOutCnt+1;
      |     set_param([gcb '/fltIntegPartK_1_Out'], 'Port', num2str(tmpOutCnt));
      |     tmpOutCnt=tmpOutCnt+1;
      |     set_param([gcb '/fltInK_1_Out'], 'Port', num2str(tmpOutCnt));
      | 
      |     set_param(gcb,'MaskEnables',{'on','on','on','off','off','off','off','off','off','off','off','off','off'});
      | 
      |     if (posblk(4) - posblk(2)) < 225
      |       height = 225;
      |       set_param(gcb,'Position',[posblk(1), posblk(2), posblk(3), posblk(2)+height])
      |     end
      |   end
      | end
      settings: RTWSystemCode=Inline
      mask Help: web([fileparts(which('ammclib_bam_S32K3xx.slx')) '/../doc/S32K3XXMCLUG.pdf'], '-browser')
      mask TypeOptions showStates: Hide (faster execution) | Show (allows debugging; connect feedback loops manually)
      mask Callback showStates:
      | maskStr=get_param(gcb,'showStates');
      | if strcmp(maskStr,'Hide (faster execution)')
      |   if strcmp(get_param([gcb '/fltPropGain'], 'BlockType'), 'Inport')
      |     autoCalcEn=get_param(gcb,'autoCalcEn');
      |     if strcmp(autoCalcEn,'on')
      |       set_param(gcb,'MaskEnables',{'on','on','on','on','on','on','on','on','on','on','on','on','off'});
      |     else
      |       set_param(gcb,'MaskEnables',{'on','on','on','off','off','off','off','on','on','on','on','on','off'});
      |     end
      |   end
      | else
      |   if strcmp(get_param([gcb '/fltPropGain'], 'BlockType'), 'Ground')
      |     set_param(gcb,'MaskEnables',{'on','on','on','off','off','off','off','off','off','off','off','off','off'});
      |   end
      | end
      mask TypeOptions resetStatesEnable: Pre-set according to the first set of inputs after reset | Clear to zero
      mask TypeOptions SampleTime: fltInErr/SampleTime | fltControllerPIpAWOut_preset/SampleTime
      mask Callback SampleTime:
      | p=Simulink.Mask.get(gcb);
      | hintText=p.getDialogControl('timeHint');
      | SampleTime=Simulink.data.evalinGlobal(bdroot,get_param(gcb,'SampleTime'));
      | SampleTime_1=str2double(get_param(gcb,'SampleTime_1'));
      | if (((SampleTime==-1) && (~contains(hintText.Prompt,'inherited'))) || ...
      |     ((SampleTime~=-1) && contains(hintText.Prompt,'inherited')) || ...
      |     ((SampleTime~=-1) && (SampleTime_1~=SampleTime)) || ...
      |     ((SampleTime_1~=-1) && contains(hintText.Prompt,'yet')))
      |   if ((SampleTime==-1) && (~contains(hintText.Prompt,'inherited')))
      |     set_param(gcb,'SampleTime_1',num2str(NaN));
      |     SampleTime_1=NaN;
      |   end
      |   if (SampleTime~=-1)
      |     set_param(gcb,'SampleTime_1',num2str(SampleTime));
      |     SampleTime_1=SampleTime;
      |   end
      |   autoCalcEn=get_param(gcb,'autoCalcEn');
      |   if strcmp(autoCalcEn,'on')
      |     p=Simulink.Mask.get(gcb);
      |     hintText=p.getDialogControl('timeHint');
      |     if SampleTime==-1
      |       SampleTime=SampleTime_1;
      |       if isnan(SampleTime)
      |         hintText.Prompt='Note: Implementation parameters cannot be calculated yet because the block''s inherited sample time is unknown. Simulink will update the sample time when you run the simulation.';
      |       else
      |         hintText.Prompt='Caution: Implementation parameters depend on inherited sample time. Make sure that the sample time of the block''s inputs corresponds to the sampling period in the target application.';
      |       end
      |     else
      |       hintText.Prompt='Caution: Implementation parameters depend on the sample time. Make sure that the simulation time step corresponds to the sampling period in the target application.';
      |     end
      |     fltPropGain_bkup=get_param(gcb,'fltPropGain');
      |     fltIntegGain_bkup=get_param(gcb,'fltIntegGain');
      |     fltLowerLimit_bkup=get_param(gcb,'fltLowerLimit');
      |     fltUpperLimit_bkup=get_param(gcb,'fltUpperLimit');
      |     pgain=Simulink.data.evalinGlobal(bdroot,get_param(gcb,'pgain'));
      |     igain=Simulink.data.evalinGlobal(bdroot,get_param(gcb,'igain'));
      |     lowerLimit=Simulink.data.evalinGlobal(bdroot,get_param(gcb,'lowerLimit'));
      |     upperLimit=Simulink.data.evalinGlobal(bdroot,get_param(gcb,'upperLimit'));
      |     if (upperLimit<=lowerLimit)
      |       warning('UpperLimit should be greater than LowerLimit.');
      |     end
      |     fltPropGain=pgain;
      |     fltIntegGain=igain*SampleTime*0.5;
      |     fltUpperLimit=upperLimit;
      |     fltLowerLimit=lowerLimit;
      |     if isnan(fltPropGain)
      |       if ~strcmp(fltPropGain_bkup,'0')
      |         set_param(gcb,'fltPropGain','0');
      |       end
      |     else
      |       tmps=num2str(fltPropGain);
      |       if ~strcmp(fltPropGain_bkup,tmps)
      |         set_param(gcb,'fltPropGain',tmps);
      |       end
      |     end
      |     if isnan(fltIntegGain)
      |       if ~strcmp(fltIntegGain_bkup,'0')
      |         set_param(gcb,'fltIntegGain','0');
      |       end
      |     else
      |       tmps=num2str(fltIntegGain);
      |       if ~strcmp(fltIntegGain_bkup,tmps)
      |         set_param(gcb,'fltIntegGain',tmps);
      |       end
      |     end
      |     if isnan(fltLowerLimit)
      |       if ~strcmp(fltLowerLimit_bkup,'0')
      |         set_param(gcb,'fltLowerLimit','0');
      |       end
      |     else
      |       tmps=num2str(fltLowerLimit);
      |       if ~strcmp(fltLowerLimit_bkup,tmps)
      |         set_param(gcb,'fltLowerLimit',tmps);
      |       end
      |     end
      |     if isnan(fltUpperLimit)
      |       if ~strcmp(fltUpperLimit_bkup,'0')
      |         set_param(gcb,'fltUpperLimit','0');
      |       end
      |     else
      |       tmps=num2str(fltUpperLimit);
      |       if ~strcmp(fltUpperLimit_bkup,tmps)
      |         set_param(gcb,'fltUpperLimit',tmps);
      |       end
      |     end
      |   end
      | end
      mask Callback pgain:
      | autoCalcEn=get_param(gcb,'autoCalcEn');
      | if strcmp(autoCalcEn,'on')
      |   SampleTime=Simulink.data.evalinGlobal(bdroot,get_param(gcb,'SampleTime'));
      |   if (SampleTime==-1)
      |     SampleTime=str2double(get_param(gcb,'SampleTime_1'));
      |   end
      |   fltPropGain_bkup=get_param(gcb,'fltPropGain');
      |   fltIntegGain_bkup=get_param(gcb,'fltIntegGain');
      |   fltLowerLimit_bkup=get_param(gcb,'fltLowerLimit');
      |   fltUpperLimit_bkup=get_param(gcb,'fltUpperLimit');
      |   pgain=Simulink.data.evalinGlobal(bdroot,get_param(gcb,'pgain'));
      |   igain=Simulink.data.evalinGlobal(bdroot,get_param(gcb,'igain'));
      |   lowerLimit=Simulink.data.evalinGlobal(bdroot,get_param(gcb,'lowerLimit'));
      |   upperLimit=Simulink.data.evalinGlobal(bdroot,get_param(gcb,'upperLimit'));
      |   if (upperLimit<=lowerLimit)
      |     warning('UpperLimit should be greater than LowerLimit.');
      |   end
      |   fltPropGain=pgain;
      |   fltIntegGain=igain*SampleTime*0.5;
      |   fltUpperLimit=upperLimit;
      |   fltLowerLimit=lowerLimit;
      |   if isnan(fltPropGain)
      |     if ~strcmp(fltPropGain_bkup,'0')
      |       set_param(gcb,'fltPropGain','0');
      |     end
      |   else
      |     tmps=num2str(fltPropGain);
      |     if ~strcmp(fltPropGain_bkup,tmps)
      |       set_param(gcb,'fltPropGain',tmps);
      |     end
      |   end
      |   if isnan(fltIntegGain)
      |     if ~strcmp(fltIntegGain_bkup,'0')
      |       set_param(gcb,'fltIntegGain','0');
      |     end
      |   else
      |     tmps=num2str(fltIntegGain);
      |     if ~strcmp(fltIntegGain_bkup,tmps)
      |       set_param(gcb,'fltIntegGain',tmps);
      |     end
      |   end
      |   if isnan(fltLowerLimit)
      |     if ~strcmp(fltLowerLimit_bkup,'0')
      |       set_param(gcb,'fltLowerLimit','0');
      |     end
      |   else
      |     tmps=num2str(fltLowerLimit);
      |     if ~strcmp(fltLowerLimit_bkup,tmps)
      |       set_param(gcb,'fltLowerLimit',tmps);
      |     end
      |   end
      |   if isnan(fltUpperLimit)
      |     if ~strcmp(fltUpperLimit_bkup,'0')
      |       set_param(gcb,'fltUpperLimit','0');
      |     end
      |   else
      |     tmps=num2str(fltUpperLimit);
      |     if ~strcmp(fltUpperLimit_bkup,tmps)
      |       set_param(gcb,'fltUpperLimit',tmps);
      |     end
      |   end
      | end
      mask Callback igain:
      | autoCalcEn=get_param(gcb,'autoCalcEn');
      | if strcmp(autoCalcEn,'on')
      |   SampleTime=Simulink.data.evalinGlobal(bdroot,get_param(gcb,'SampleTime'));
      |   if (SampleTime==-1)
      |     SampleTime=str2double(get_param(gcb,'SampleTime_1'));
      |   end
      |   fltPropGain_bkup=get_param(gcb,'fltPropGain');
      |   fltIntegGain_bkup=get_param(gcb,'fltIntegGain');
      |   fltLowerLimit_bkup=get_param(gcb,'fltLowerLimit');
      |   fltUpperLimit_bkup=get_param(gcb,'fltUpperLimit');
      |   pgain=Simulink.data.evalinGlobal(bdroot,get_param(gcb,'pgain'));
      |   igain=Simulink.data.evalinGlobal(bdroot,get_param(gcb,'igain'));
      |   lowerLimit=Simulink.data.evalinGlobal(bdroot,get_param(gcb,'lowerLimit'));
      |   upperLimit=Simulink.data.evalinGlobal(bdroot,get_param(gcb,'upperLimit'));
      |   if (upperLimit<=lowerLimit)
      |     warning('UpperLimit should be greater than LowerLimit.');
      |   end
      |   fltPropGain=pgain;
      |   fltIntegGain=igain*SampleTime*0.5;
      |   fltUpperLimit=upperLimit;
      |   fltLowerLimit=lowerLimit;
      |   if isnan(fltPropGain)
      |     if ~strcmp(fltPropGain_bkup,'0')
      |       set_param(gcb,'fltPropGain','0');
      |     end
      |   else
      |     tmps=num2str(fltPropGain);
      |     if ~strcmp(fltPropGain_bkup,tmps)
      |       set_param(gcb,'fltPropGain',tmps);
      |     end
      |   end
      |   if isnan(fltIntegGain)
      |     if ~strcmp(fltIntegGain_bkup,'0')
      |       set_param(gcb,'fltIntegGain','0');
      |     end
      |   else
      |     tmps=num2str(fltIntegGain);
      |     if ~strcmp(fltIntegGain_bkup,tmps)
      |       set_param(gcb,'fltIntegGain',tmps);
      |     end
      |   end
      |   if isnan(fltLowerLimit)
      |     if ~strcmp(fltLowerLimit_bkup,'0')
      |       set_param(gcb,'fltLowerLimit','0');
      |     end
      |   else
      |     tmps=num2str(fltLowerLimit);
      |     if ~strcmp(fltLowerLimit_bkup,tmps)
      |       set_param(gcb,'fltLowerLimit',tmps);
      |     end
      |   end
      |   if isnan(fltUpperLimit)
      |     if ~strcmp(fltUpperLimit_bkup,'0')
      |       set_param(gcb,'fltUpperLimit','0');
      |     end
      |   else
      |     tmps=num2str(fltUpperLimit);
      |     if ~strcmp(fltUpperLimit_bkup,tmps)
      |       set_param(gcb,'fltUpperLimit',tmps);
      |     end
      |   end
      | end
      mask Callback lowerLimit:
      | autoCalcEn=get_param(gcb,'autoCalcEn');
      | if strcmp(autoCalcEn,'on')
      |   SampleTime=Simulink.data.evalinGlobal(bdroot,get_param(gcb,'SampleTime'));
      |   if (SampleTime==-1)
      |     SampleTime=str2double(get_param(gcb,'SampleTime_1'));
      |   end
      |   fltPropGain_bkup=get_param(gcb,'fltPropGain');
      |   fltIntegGain_bkup=get_param(gcb,'fltIntegGain');
      |   fltLowerLimit_bkup=get_param(gcb,'fltLowerLimit');
      |   fltUpperLimit_bkup=get_param(gcb,'fltUpperLimit');
      |   pgain=Simulink.data.evalinGlobal(bdroot,get_param(gcb,'pgain'));
      |   igain=Simulink.data.evalinGlobal(bdroot,get_param(gcb,'igain'));
      |   lowerLimit=Simulink.data.evalinGlobal(bdroot,get_param(gcb,'lowerLimit'));
      |   upperLimit=Simulink.data.evalinGlobal(bdroot,get_param(gcb,'upperLimit'));
      |   if (upperLimit<=lowerLimit)
      |     warning('UpperLimit should be greater than LowerLimit.');
      |   end
      |   fltPropGain=pgain;
      |   fltIntegGain=igain*SampleTime*0.5;
      |   fltUpperLimit=upperLimit;
      |   fltLowerLimit=lowerLimit;
      |   if isnan(fltPropGain)
      |     if ~strcmp(fltPropGain_bkup,'0')
      |       set_param(gcb,'fltPropGain','0');
      |     end
      |   else
      |     tmps=num2str(fltPropGain);
      |     if ~strcmp(fltPropGain_bkup,tmps)
      |       set_param(gcb,'fltPropGain',tmps);
      |     end
      |   end
      |   if isnan(fltIntegGain)
      |     if ~strcmp(fltIntegGain_bkup,'0')
      |       set_param(gcb,'fltIntegGain','0');
      |     end
      |   else
      |     tmps=num2str(fltIntegGain);
      |     if ~strcmp(fltIntegGain_bkup,tmps)
      |       set_param(gcb,'fltIntegGain',tmps);
      |     end
      |   end
      |   if isnan(fltLowerLimit)
      |     if ~strcmp(fltLowerLimit_bkup,'0')
      |       set_param(gcb,'fltLowerLimit','0');
      |     end
      |   else
      |     tmps=num2str(fltLowerLimit);
      |     if ~strcmp(fltLowerLimit_bkup,tmps)
      |       set_param(gcb,'fltLowerLimit',tmps);
      |     end
      |   end
      |   if isnan(fltUpperLimit)
      |     if ~strcmp(fltUpperLimit_bkup,'0')
      |       set_param(gcb,'fltUpperLimit','0');
      |     end
      |   else
      |     tmps=num2str(fltUpperLimit);
      |     if ~strcmp(fltUpperLimit_bkup,tmps)
      |       set_param(gcb,'fltUpperLimit',tmps);
      |     end
      |   end
      | end
      mask Callback upperLimit:
      | autoCalcEn=get_param(gcb,'autoCalcEn');
      | if strcmp(autoCalcEn,'on')
      |   SampleTime=Simulink.data.evalinGlobal(bdroot,get_param(gcb,'SampleTime'));
      |   if (SampleTime==-1)
      |     SampleTime=str2double(get_param(gcb,'SampleTime_1'));
      |   end
      |   fltPropGain_bkup=get_param(gcb,'fltPropGain');
      |   fltIntegGain_bkup=get_param(gcb,'fltIntegGain');
      |   fltLowerLimit_bkup=get_param(gcb,'fltLowerLimit');
      |   fltUpperLimit_bkup=get_param(gcb,'fltUpperLimit');
      |   pgain=Simulink.data.evalinGlobal(bdroot,get_param(gcb,'pgain'));
      |   igain=Simulink.data.evalinGlobal(bdroot,get_param(gcb,'igain'));
      |   lowerLimit=Simulink.data.evalinGlobal(bdroot,get_param(gcb,'lowerLimit'));
      |   upperLimit=Simulink.data.evalinGlobal(bdroot,get_param(gcb,'upperLimit'));
      |   if (upperLimit<=lowerLimit)
      |     warning('UpperLimit should be greater than LowerLimit.');
      |   end
      |   fltPropGain=pgain;
      |   fltIntegGain=igain*SampleTime*0.5;
      |   fltUpperLimit=upperLimit;
      |   fltLowerLimit=lowerLimit;
      |   if isnan(fltPropGain)
      |     if ~strcmp(fltPropGain_bkup,'0')
      |       set_param(gcb,'fltPropGain','0');
      |     end
      |   else
      |     tmps=num2str(fltPropGain);
      |     if ~strcmp(fltPropGain_bkup,tmps)
      |       set_param(gcb,'fltPropGain',tmps);
      |     end
      |   end
      |   if isnan(fltIntegGain)
      |     if ~strcmp(fltIntegGain_bkup,'0')
      |       set_param(gcb,'fltIntegGain','0');
      |     end
      |   else
      |     tmps=num2str(fltIntegGain);
      |     if ~strcmp(fltIntegGain_bkup,tmps)
      |       set_param(gcb,'fltIntegGain',tmps);
      |     end
      |   end
      |   if isnan(fltLowerLimit)
      |     if ~strcmp(fltLowerLimit_bkup,'0')
      |       set_param(gcb,'fltLowerLimit','0');
      |     end
      |   else
      |     tmps=num2str(fltLowerLimit);
      |     if ~strcmp(fltLowerLimit_bkup,tmps)
      |       set_param(gcb,'fltLowerLimit',tmps);
      |     end
      |   end
      |   if isnan(fltUpperLimit)
      |     if ~strcmp(fltUpperLimit_bkup,'0')
      |       set_param(gcb,'fltUpperLimit','0');
      |     end
      |   else
      |     tmps=num2str(fltUpperLimit);
      |     if ~strcmp(fltUpperLimit_bkup,tmps)
      |       set_param(gcb,'fltUpperLimit',tmps);
      |     end
      |   end
      | end
      mask Callback autoCalcEn:
      | maskStr=get_param(gcb,'showStates');
      | if strcmp(maskStr,'Hide (faster execution)')
      |   p=Simulink.Mask.get(gcb);
      |   autoCalcEn=get_param(gcb,'autoCalcEn');
      |   hintText=p.getDialogControl('timeHint');
      |   if strcmp(autoCalcEn,'on')
      |     param=p.getParameter('upperLimit');
      |     if strcmp(param.Enabled,'off')
      |       SampleTime=Simulink.data.evalinGlobal(bdroot,get_param(gcb,'SampleTime'));
      |       if SampleTime==-1
      |         SampleTime=str2double(get_param(gcb,'SampleTime_1'));
      |         if isnan(SampleTime)
      |           hintText.Prompt=['Note: Implementation parameters cannot be calculated yet because the block''s inherited sample time is unknown. Simulink will update the sample time when you run the simulation.'];
      |         else
      |           hintText.Prompt=['Caution: Implementation parameters depend on inherited sample time. Make sure that the sample time of the block''s inputs corresponds to the sampling period in the target application.'];
      |         end
      |       else
      |         hintText.Prompt='Caution: Implementation parameters depend on the sample time. Make sure that the simulation time step corresponds to the sampling period in the target application.';
      |       end
      |       p=Simulink.Mask.get(gcb);
      |       param=p.getParameter('pgain');
      |       param.set('Enabled','on');
      |       param=p.getParameter('igain');
      |       param.set('Enabled','on');
      |       param=p.getParameter('lowerLimit');
      |       param.set('Enabled','on');
      |       param=p.getParameter('upperLimit');
      |       param.set('Enabled','on');
      |     else
      |       SampleTime=Simulink.data.evalinGlobal(bdroot,get_param(gcb,'SampleTime'));
      |       if SampleTime==-1
      |         SampleTime=str2double(get_param(gcb,'SampleTime_1'));
      |       end
      |     end
      |     fltPropGain_bkup=get_param(gcb,'fltPropGain');
      |     fltIntegGain_bkup=get_param(gcb,'fltIntegGain');
      |     fltLowerLimit_bkup=get_param(gcb,'fltLowerLimit');
      |     fltUpperLimit_bkup=get_param(gcb,'fltUpperLimit');
      |     pgain=Simulink.data.evalinGlobal(bdroot,get_param(gcb,'pgain'));
      |     igain=Simulink.data.evalinGlobal(bdroot,get_param(gcb,'igain'));
      |     lowerLimit=Simulink.data.evalinGlobal(bdroot,get_param(gcb,'lowerLimit'));
      |     upperLimit=Simulink.data.evalinGlobal(bdroot,get_param(gcb,'upperLimit'));
      |     if (upperLimit<=lowerLimit)
      |       warning('UpperLimit should be greater than LowerLimit.');
      |     end
      |     fltPropGain=pgain;
      |     fltIntegGain=igain*SampleTime*0.5;
      |     fltUpperLimit=upperLimit;
      |     fltLowerLimit=lowerLimit;
      |     if isnan(fltPropGain)
      |       if ~strcmp(fltPropGain_bkup,'0')
      |         set_param(gcb,'fltPropGain','0');
      |       end
      |     else
      |       tmps=num2str(fltPropGain);
      |       if ~strcmp(fltPropGain_bkup,tmps)
      |         set_param(gcb,'fltPropGain',tmps);
      |       end
      |     end
      |     if isnan(fltIntegGain)
      |       if ~strcmp(fltIntegGain_bkup,'0')
      |         set_param(gcb,'fltIntegGain','0');
      |       end
      |     else
      |       tmps=num2str(fltIntegGain);
      |       if ~strcmp(fltIntegGain_bkup,tmps)
      |         set_param(gcb,'fltIntegGain',tmps);
      |       end
      |     end
      |     if isnan(fltLowerLimit)
      |       if ~strcmp(fltLowerLimit_bkup,'0')
      |         set_param(gcb,'fltLowerLimit','0');
      |       end
      |     else
      |       tmps=num2str(fltLowerLimit);
      |       if ~strcmp(fltLowerLimit_bkup,tmps)
      |         set_param(gcb,'fltLowerLimit',tmps);
      |       end
      |     end
      |     if isnan(fltUpperLimit)
      |       if ~strcmp(fltUpperLimit_bkup,'0')
      |         set_param(gcb,'fltUpperLimit','0');
      |       end
      |     else
      |       tmps=num2str(fltUpperLimit);
      |       if ~strcmp(fltUpperLimit_bkup,tmps)
      |         set_param(gcb,'fltUpperLimit',tmps);
      |       end
      |     end
      |   else
      |     param=p.getParameter('upperLimit');
      |     if strcmp(param.Enabled,'on')
      |       hintText.Prompt='Caution: Implementation parameters are fixed.';
      |       p=Simulink.Mask.get(gcb);
      |       param=p.getParameter('pgain');
      |       param.set('Enabled','off');
      |       param=p.getParameter('igain');
      |       param.set('Enabled','off');
      |       param=p.getParameter('lowerLimit');
      |       param.set('Enabled','off');
      |       param=p.getParameter('upperLimit');
      |       param.set('Enabled','off');
      |     end
      |   end
      | end
      mask DialogControl CompBut Prompt: Recalculate sample times
      mask DialogControl CompBut Tooltip: Simulink updates the sample times of all blocks when the simulation is run. This button will update the sample times now.
      mask DialogControl CompBut Callback:
      | btn=questdlg('This will apply all changes in all open dialog boxes and update the schematic. Do you want to proceed?','Apply all changes','Continue','Cancel','Continue');
      | if strcmp(btn,'Continue')
      |   dlgs=DAStudio.ToolRoot.getOpenDialogs;
      |   for i=1:length(dlgs)
      |     dlgs(i).apply;
      |   end
      |   try
      |     SampleTime_1=str2double(get_param(gcb,'SampleTime_1'));
      |     ts=Simulink.Block.getSampleTimes(gcb);
      |     ts=ts(1).Value(1);
      |     if (SampleTime_1 ~= ts)
      |       SampleTime_1=ts;
      |       set_param(gcb,'SampleTime_1',num2str(ts));
      |       autoCalcEn=get_param(gcb,'autoCalcEn');
      |       if strcmp(autoCalcEn,'on')
      |         SampleTime=Simulink.data.evalinGlobal(bdroot,get_param(gcb,'SampleTime'));
      |         p=Simulink.Mask.get(gcb);
      |         hintText=p.getDialogControl('timeHint');
      |         if SampleTime==-1
      |           SampleTime=SampleTime_1;
      |           hintText.Prompt='Caution: Implementation parameters depend on inherited sample time. Make sure that the sample time of the block''s inputs corresponds to the sampling period in the target application.';
      |         else
      |           hintText.Prompt='Caution: Implementation parameters depend on the sample time. Make sure that the simulation time step corresponds to the sampling period in the target application.';
      |         end
      |         fltPropGain_bkup=get_param(gcb,'fltPropGain');
      |         fltIntegGain_bkup=get_param(gcb,'fltIntegGain');
      |         fltLowerLimit_bkup=get_param(gcb,'fltLowerLimit');
      |         fltUpperLimit_bkup=get_param(gcb,'fltUpperLimit');
      |         pgain=Simulink.data.evalinGlobal(bdroot,get_param(gcb,'pgain'));
      |         igain=Simulink.data.evalinGlobal(bdroot,get_param(gcb,'igain'));
      |         lowerLimit=Simulink.data.evalinGlobal(bdroot,get_param(gcb,'lowerLimit'));
      |         upperLimit=Simulink.data.evalinGlobal(bdroot,get_param(gcb,'upperLimit'));
      |         if (upperLimit<=lowerLimit)
      |           warning('UpperLimit should be greater than LowerLimit.');
      |         end
      |         fltPropGain=pgain;
      |         fltIntegGain=igain*SampleTime*0.5;
      |         fltUpperLimit=upperLimit;
      |         fltLowerLimit=lowerLimit;
      |         if isnan(fltPropGain)
      |           if ~strcmp(fltPropGain_bkup,'0')
      |             set_param(gcb,'fltPropGain','0');
      |           end
      |         else
      |           tmps=num2str(fltPropGain);
      |           if ~strcmp(fltPropGain_bkup,tmps)
      |             set_param(gcb,'fltPropGain',tmps);
      |           end
      |         end
      |         if isnan(fltIntegGain)
      |           if ~strcmp(fltIntegGain_bkup,'0')
      |             set_param(gcb,'fltIntegGain','0');
      |           end
      |         else
      |           tmps=num2str(fltIntegGain);
      |           if ~strcmp(fltIntegGain_bkup,tmps)
      |             set_param(gcb,'fltIntegGain',tmps);
      |           end
      |         end
      |         if isnan(fltLowerLimit)
      |           if ~strcmp(fltLowerLimit_bkup,'0')
      |             set_param(gcb,'fltLowerLimit','0');
      |           end
      |         else
      |           tmps=num2str(fltLowerLimit);
      |           if ~strcmp(fltLowerLimit_bkup,tmps)
      |             set_param(gcb,'fltLowerLimit',tmps);
      |           end
      |         end
      |         if isnan(fltUpperLimit)
      |           if ~strcmp(fltUpperLimit_bkup,'0')
      |             set_param(gcb,'fltUpperLimit','0');
      |           end
      |         else
      |           tmps=num2str(fltUpperLimit);
      |           if ~strcmp(fltUpperLimit_bkup,tmps)
      |             set_param(gcb,'fltUpperLimit',tmps);
      |           end
      |         end
      |       end
      |     end
      |   catch
      |    warning(['Sample time cannot be calculated for the block ' gcb])
      |   end
      | end
      mask DialogControl timeHint Prompt: Note: Implementation parameters cannot be calculated yet because the block's inherited sample time is unknown. Simulink will update the sample time when you run the simulation.
      mask Display:
      | color('black');
      | pos = get_param(gcb, 'Position');
      | width = pos(3) - pos(1);
      | height = pos(4) - pos(2);
      | tX=width/2;
      | tY=height - 25;
      | color('black');
      | text(tX,tY, 'GFLIB_ControllerPIpAW_FLT', 'horizontalAlignment', 'center');
      | if showStates == 2
      |   color('red');
      |   text(tX,tY - 20, ['debugging mode' char(13) char(10) '(limited performance)'], 'horizontalAlignment', 'center');
      | end
  GFLIB_ControllerPIp_FLT : Subsystem  StartFcn=|  TreatAsAtomicUnit=on  mask(GFLIB_ControllerPIp_FLT){showStates=Hide (faster execution), resetStatesEnable=Pre-set according to the first set of inputs after reset, SampleTime=-1, pgain=5, igain=0.5, autoCalcEn=on, fltPropGain=0, fltIntegGain=0, SampleTime_1=NaN}
      | ts=get_param(gcb,'CompiledSampleTime');
      | if iscell(ts)
      |   ts=ts{1};
      |   if iscell(ts)
      |     ts=ts{1};
      |   end
      | end
      | ts=ts(1);
      | set_param(gcb,'SampleTime_1',num2str(ts));
      | p=Simulink.Mask.get(gcb);
      | hintText=p.getDialogControl('timeHint');
      | SampleTime=Simulink.data.evalinGlobal(bdroot,get_param(gcb,'SampleTime'));
      | p=Simulink.Mask.get(gcb);
      | autoCalcEn=get_param(gcb,'autoCalcEn');
      | if strcmp(autoCalcEn,'on')
      |   if SampleTime==-1
      |     hintText.Prompt='Caution: Implementation parameters depend on inherited sample time. Make sure that the sample time of the block''s inputs corresponds to the sampling period in the target application.';
      |   else
      |     hintText.Prompt='Caution: Implementation parameters depend on the sample time. Make sure that the simulation time step corresponds to the sampling period in the target application.';
      |   end
      |   SampleTime=ts;
      |   fltPropGain_bkup=get_param(gcb,'fltPropGain');
      |   fltIntegGain_bkup=get_param(gcb,'fltIntegGain');
      |   pgain=Simulink.data.evalinGlobal(bdroot,get_param(gcb,'pgain'));
      |   igain=Simulink.data.evalinGlobal(bdroot,get_param(gcb,'igain'));
      |   fltPropGain=pgain;
      |   fltIntegGain=igain*SampleTime*0.5;
      |   if isnan(fltPropGain)
      |     if ~strcmp(fltPropGain_bkup,'0')
      |       set_param(gcb,'fltPropGain','0');
      |     end
      |   else
      |     tmps=num2str(fltPropGain);
      |     if ~strcmp(fltPropGain_bkup,tmps)
      |       set_param(gcb,'fltPropGain',tmps);
      |     end
      |   end
      |   if isnan(fltIntegGain)
      |     if ~strcmp(fltIntegGain_bkup,'0')
      |       set_param(gcb,'fltIntegGain','0');
      |     end
      |   else
      |     tmps=num2str(fltIntegGain);
      |     if ~strcmp(fltIntegGain_bkup,tmps)
      |       set_param(gcb,'fltIntegGain',tmps);
      |     end
      |   end
      | end
      mask prompts: showStates "Show internal states:"; resetStatesEnable "Internal state after reset:"; SampleTime "Sample time (-1 for inherited):"; pgain "Proportional gain (P):"; igain "Integral gain (I):"; autoCalcEn "Calculate implementation parameters from physical parameters"; fltPropGain "fltPropGain (Proportional gain):"; fltIntegGain "fltIntegGain (Integral gain):"; SampleTime_1 "Discrete sample time:"
      mask help: Parallel form discrete-time PI controller without anti-windup in single precision floating-point implementation. This block supports re-initialization of the internal state during simulation. If the block is reset, the controller's output will be aligned with the input fltControllerPIpOut_preset. Refer to the AMMCLIB User's Guide for further details.
      mask init:
      | ddName = get_param(bdroot,'DataDictionary');
      | if length(ddName)==0
      |   set_param(bdroot,'DataDictionary','ammclib_types.sldd');
      | else
      |   dd = Simulink.data.dictionary.open(ddName);
      |   data = getSection(dd,'Design Data');
      |   if ~exist(data,'SWLIBS_2Syst_F16')
      |     addDataSource(dd,'ammclib_types.sldd');
      |     saveChanges(dd);
      |   end
      | end
      | 
      | if showStates == 1
      |   % hidden state variables
      |   if strcmp(get_param([gcb '/fltPropGain'], 'BlockType'), 'Inport')
      |     posblk = get_param(gcb, 'Position');
      | 
      |     pos = get_param([gcb, '/fltPropGain'], 'Position');
      |     orient = get_param([gcb, '/fltPropGain'], 'Orientation');
      |     delete_block([gcb, '/fltPropGain']);
      |     add_block('built-in/Ground', [gcb, '/fltPropGain'], 'Position', pos, 'Orientation', orient);
      | 
      |     pos = get_param([gcb, '/fltIntegGain'], 'Position');
      |     orient = get_param([gcb, '/fltIntegGain'], 'Orientation');
      |     delete_block([gcb, '/fltIntegGain']);
      |     add_block('built-in/Ground', [gcb, '/fltIntegGain'], 'Position', pos, 'Orientation', orient);
      | 
      |     pos = get_param([gcb, '/fltIntegPartK_1'], 'Position');
      |     orient = get_param([gcb, '/fltIntegPartK_1'], 'Orientation');
      |     delete_block([gcb, '/fltIntegPartK_1']);
      |     add_block('built-in/Ground', [gcb, '/fltIntegPartK_1'], 'Position', pos, 'Orientation', orient);
      | 
      |     pos = get_param([gcb, '/fltInK_1'], 'Position');
      |     orient = get_param([gcb, '/fltInK_1'], 'Orientation');
      |     delete_block([gcb, '/fltInK_1']);
      |     add_block('built-in/Ground', [gcb, '/fltInK_1'], 'Position', pos, 'Orientation', orient);
      | 
      | 
      |     pmask=Simulink.Mask.get(gcb);
      |     pctrl=pmask.getParameter('SampleTime');
      |     pctrl.set('TypeOptions',{'fltInErr/SampleTime','fltControllerPIpOut_preset/SampleTime'});
      | 
      |     pos = get_param([gcb '/fltIntegPartK_1_Out'], 'Position');
      |     orient = get_param([gcb '/fltIntegPartK_1_Out'], 'Orientation');
      |     delete_block([gcb '/fltIntegPartK_1_Out']);
      |     add_block('built-in/Terminator', [gcb '/fltIntegPartK_1_Out'], 'Position', pos, 'Orientation', orient);
      | 
      |     pos = get_param([gcb '/fltInK_1_Out'], 'Position');
      |     orient = get_param([gcb '/fltInK_1_Out'], 'Orientation');
      |     delete_block([gcb '/fltInK_1_Out']);
      |     add_block('built-in/Terminator', [gcb '/fltInK_1_Out'], 'Position', pos, 'Orientation', orient);
      | 
      |     set_param([gcb '/fltInErr'], 'Port', '1');
      |     set_param([gcb '/fltControllerPIpOut_preset'], 'Port', '2');
      | 
      |     tmpOutCnt=0;
      |     tmpOutCnt=tmpOutCnt+1;
      |     set_param([gcb '/fltOut'], 'Port', num2str(tmpOutCnt));
      | 
      |     autoCalcEn=get_param(gcb,'autoCalcEn');
      |     if strcmp(autoCalcEn,'on')
      |       set_param(gcb,'MaskEnables',{'on','on','on','on','on','on','on','on','off'});
      |     else
      |       set_param(gcb,'MaskEnables',{'on','on','on','off','off','on','on','on','off'});
      |     end
      | 
      |     if (posblk(4) - posblk(2)) > 75
      |       height = 75;
      |       set_param(gcb,'Position',[posblk(1), posblk(2), posblk(3), posblk(2)+height])
      |     end
      |   end
      | else
      |   % shown state variables
      |   if strcmp(get_param([gcb '/fltPropGain'], 'BlockType'), 'Ground')
      |     posblk = get_param(gcb, 'Position');
      | 
      |     pos = get_param([gcb, '/fltPropGain'], 'Position');
      |     orient = get_param([gcb, '/fltPropGain'], 'Orientation');
      |     delete_block([gcb, '/fltPropGain']);
      |     add_block('built-in/Inport', [gcb, '/fltPropGain'], 'Position', pos, 'Orientation', orient, 'OutDataTypeStr', 'single');
      | 
      |     pos = get_param([gcb, '/fltIntegGain'], 'Position');
      |     orient = get_param([gcb, '/fltIntegGain'], 'Orientation');
      |     delete_block([gcb, '/fltIntegGain']);
      |     add_block('built-in/Inport', [gcb, '/fltIntegGain'], 'Position', pos, 'Orientation', orient, 'OutDataTypeStr', 'single');
      | 
      |     pos = get_param([gcb, '/fltIntegPartK_1'], 'Position');
      |     orient = get_param([gcb, '/fltIntegPartK_1'], 'Orientation');
      |     delete_block([gcb, '/fltIntegPartK_1']);
      |     add_block('built-in/Inport', [gcb, '/fltIntegPartK_1'], 'Position', pos, 'Orientation', orient, 'OutDataTypeStr', 'single');
      | 
      |     pos = get_param([gcb, '/fltInK_1'], 'Position');
      |     orient = get_param([gcb, '/fltInK_1'], 'Orientation');
      |     delete_block([gcb, '/fltInK_1']);
      |     add_block('built-in/Inport', [gcb, '/fltInK_1'], 'Position', pos, 'Orientation', orient, 'OutDataTypeStr', 'single');
      | 
      | 
      | 
      |     pos = get_param([gcb '/fltIntegPartK_1_Out'], 'Position');
      |     orient = get_param([gcb '/fltIntegPartK_1_Out'], 'Orientation');
      |     delete_block([gcb '/fltIntegPartK_1_Out']);
      |     add_block('built-in/Outport', [gcb '/fltIntegPartK_1_Out'], 'Position', pos, 'Orientation', orient);
      | 
      |     pos = get_param([gcb '/fltInK_1_Out'], 'Position');
      |     orient = get_param([gcb '/fltInK_1_Out'], 'Orientation');
      |     delete_block([gcb '/fltInK_1_Out']);
      |     add_block('built-in/Outport', [gcb '/fltInK_1_Out'], 'Position', pos, 'Orientation', orient);
      | 
      | 
      |     pmask=Simulink.Mask.get(gcb);
      |     pctrl=pmask.getParameter('SampleTime');
      |     pctrl.set('TypeOptions',{'fltInErr/SampleTime','fltControllerPIpOut_preset/SampleTime','fltPropGain/SampleTime','fltIntegGain/SampleTime','fltIntegPartK_1/SampleTime','fltInK_1/SampleTime'});
      | 
      |     set_param([gcb '/fltInErr'], 'Port', '1');
      |     set_param([gcb '/fltControllerPIpOut_preset'], 'Port', '2');
      |     set_param([gcb '/fltPropGain'], 'Port', '3');
      |     set_param([gcb '/fltIntegGain'], 'Port', '4');
      |     set_param([gcb '/fltIntegPartK_1'], 'Port', '5');
      |     set_param([gcb '/fltInK_1'], 'Port', '6');
      | 
      |     tmpOutCnt=0;
      |     tmpOutCnt=tmpOutCnt+1;
      |     set_param([gcb '/fltOut'], 'Port', num2str(tmpOutCnt));
      |     tmpOutCnt=tmpOutCnt+1;
      |     set_param([gcb '/fltIntegPartK_1_Out'], 'Port', num2str(tmpOutCnt));
      |     tmpOutCnt=tmpOutCnt+1;
      |     set_param([gcb '/fltInK_1_Out'], 'Port', num2str(tmpOutCnt));
      | 
      |     set_param(gcb,'MaskEnables',{'on','on','on','off','off','off','off','off','off'});
      | 
      |     if (posblk(4) - posblk(2)) < 175
      |       height = 175;
      |       set_param(gcb,'Position',[posblk(1), posblk(2), posblk(3), posblk(2)+height])
      |     end
      |   end
      | end
      settings: RTWSystemCode=Inline
      mask Help: web([fileparts(which('ammclib_bam_S32K3xx.slx')) '/../doc/S32K3XXMCLUG.pdf'], '-browser')
      mask TypeOptions showStates: Hide (faster execution) | Show (allows debugging; connect feedback loops manually)
      mask Callback showStates:
      | maskStr=get_param(gcb,'showStates');
      | if strcmp(maskStr,'Hide (faster execution)')
      |   if strcmp(get_param([gcb '/fltPropGain'], 'BlockType'), 'Inport')
      |     autoCalcEn=get_param(gcb,'autoCalcEn');
      |     if strcmp(autoCalcEn,'on')
      |       set_param(gcb,'MaskEnables',{'on','on','on','on','on','on','on','on','off'});
      |     else
      |       set_param(gcb,'MaskEnables',{'on','on','on','off','off','on','on','on','off'});
      |     end
      |   end
      | else
      |   if strcmp(get_param([gcb '/fltPropGain'], 'BlockType'), 'Ground')
      |     set_param(gcb,'MaskEnables',{'on','on','on','off','off','off','off','off','off'});
      |   end
      | end
      mask TypeOptions resetStatesEnable: Pre-set according to the first set of inputs after reset | Clear to zero
      mask TypeOptions SampleTime: fltInErr/SampleTime | fltControllerPIpOut_preset/SampleTime
      mask Callback SampleTime:
      | p=Simulink.Mask.get(gcb);
      | hintText=p.getDialogControl('timeHint');
      | SampleTime=Simulink.data.evalinGlobal(bdroot,get_param(gcb,'SampleTime'));
      | SampleTime_1=str2double(get_param(gcb,'SampleTime_1'));
      | if (((SampleTime==-1) && (~contains(hintText.Prompt,'inherited'))) || ...
      |     ((SampleTime~=-1) && contains(hintText.Prompt,'inherited')) || ...
      |     ((SampleTime~=-1) && (SampleTime_1~=SampleTime)) || ...
      |     ((SampleTime_1~=-1) && contains(hintText.Prompt,'yet')))
      |   if ((SampleTime==-1) && (~contains(hintText.Prompt,'inherited')))
      |     set_param(gcb,'SampleTime_1',num2str(NaN));
      |     SampleTime_1=NaN;
      |   end
      |   if (SampleTime~=-1)
      |     set_param(gcb,'SampleTime_1',num2str(SampleTime));
      |     SampleTime_1=SampleTime;
      |   end
      |   autoCalcEn=get_param(gcb,'autoCalcEn');
      |   if strcmp(autoCalcEn,'on')
      |     p=Simulink.Mask.get(gcb);
      |     hintText=p.getDialogControl('timeHint');
      |     if SampleTime==-1
      |       SampleTime=SampleTime_1;
      |       if isnan(SampleTime)
      |         hintText.Prompt='Note: Implementation parameters cannot be calculated yet because the block''s inherited sample time is unknown. Simulink will update the sample time when you run the simulation.';
      |       else
      |         hintText.Prompt='Caution: Implementation parameters depend on inherited sample time. Make sure that the sample time of the block''s inputs corresponds to the sampling period in the target application.';
      |       end
      |     else
      |       hintText.Prompt='Caution: Implementation parameters depend on the sample time. Make sure that the simulation time step corresponds to the sampling period in the target application.';
      |     end
      |     fltPropGain_bkup=get_param(gcb,'fltPropGain');
      |     fltIntegGain_bkup=get_param(gcb,'fltIntegGain');
      |     pgain=Simulink.data.evalinGlobal(bdroot,get_param(gcb,'pgain'));
      |     igain=Simulink.data.evalinGlobal(bdroot,get_param(gcb,'igain'));
      |     fltPropGain=pgain;
      |     fltIntegGain=igain*SampleTime*0.5;
      |     if isnan(fltPropGain)
      |       if ~strcmp(fltPropGain_bkup,'0')
      |         set_param(gcb,'fltPropGain','0');
      |       end
      |     else
      |       tmps=num2str(fltPropGain);
      |       if ~strcmp(fltPropGain_bkup,tmps)
      |         set_param(gcb,'fltPropGain',tmps);
      |       end
      |     end
      |     if isnan(fltIntegGain)
      |       if ~strcmp(fltIntegGain_bkup,'0')
      |         set_param(gcb,'fltIntegGain','0');
      |       end
      |     else
      |       tmps=num2str(fltIntegGain);
      |       if ~strcmp(fltIntegGain_bkup,tmps)
      |         set_param(gcb,'fltIntegGain',tmps);
      |       end
      |     end
      |   end
      | end
      mask Callback pgain:
      | autoCalcEn=get_param(gcb,'autoCalcEn');
      | if strcmp(autoCalcEn,'on')
      |   SampleTime=Simulink.data.evalinGlobal(bdroot,get_param(gcb,'SampleTime'));
      |   if (SampleTime==-1)
      |     SampleTime=str2double(get_param(gcb,'SampleTime_1'));
      |   end
      |   fltPropGain_bkup=get_param(gcb,'fltPropGain');
      |   fltIntegGain_bkup=get_param(gcb,'fltIntegGain');
      |   pgain=Simulink.data.evalinGlobal(bdroot,get_param(gcb,'pgain'));
      |   igain=Simulink.data.evalinGlobal(bdroot,get_param(gcb,'igain'));
      |   fltPropGain=pgain;
      |   fltIntegGain=igain*SampleTime*0.5;
      |   if isnan(fltPropGain)
      |     if ~strcmp(fltPropGain_bkup,'0')
      |       set_param(gcb,'fltPropGain','0');
      |     end
      |   else
      |     tmps=num2str(fltPropGain);
      |     if ~strcmp(fltPropGain_bkup,tmps)
      |       set_param(gcb,'fltPropGain',tmps);
      |     end
      |   end
      |   if isnan(fltIntegGain)
      |     if ~strcmp(fltIntegGain_bkup,'0')
      |       set_param(gcb,'fltIntegGain','0');
      |     end
      |   else
      |     tmps=num2str(fltIntegGain);
      |     if ~strcmp(fltIntegGain_bkup,tmps)
      |       set_param(gcb,'fltIntegGain',tmps);
      |     end
      |   end
      | end
      mask Callback igain:
      | autoCalcEn=get_param(gcb,'autoCalcEn');
      | if strcmp(autoCalcEn,'on')
      |   SampleTime=Simulink.data.evalinGlobal(bdroot,get_param(gcb,'SampleTime'));
      |   if (SampleTime==-1)
      |     SampleTime=str2double(get_param(gcb,'SampleTime_1'));
      |   end
      |   fltPropGain_bkup=get_param(gcb,'fltPropGain');
      |   fltIntegGain_bkup=get_param(gcb,'fltIntegGain');
      |   pgain=Simulink.data.evalinGlobal(bdroot,get_param(gcb,'pgain'));
      |   igain=Simulink.data.evalinGlobal(bdroot,get_param(gcb,'igain'));
      |   fltPropGain=pgain;
      |   fltIntegGain=igain*SampleTime*0.5;
      |   if isnan(fltPropGain)
      |     if ~strcmp(fltPropGain_bkup,'0')
      |       set_param(gcb,'fltPropGain','0');
      |     end
      |   else
      |     tmps=num2str(fltPropGain);
      |     if ~strcmp(fltPropGain_bkup,tmps)
      |       set_param(gcb,'fltPropGain',tmps);
      |     end
      |   end
      |   if isnan(fltIntegGain)
      |     if ~strcmp(fltIntegGain_bkup,'0')
      |       set_param(gcb,'fltIntegGain','0');
      |     end
      |   else
      |     tmps=num2str(fltIntegGain);
      |     if ~strcmp(fltIntegGain_bkup,tmps)
      |       set_param(gcb,'fltIntegGain',tmps);
      |     end
      |   end
      | end
      mask Callback autoCalcEn:
      | maskStr=get_param(gcb,'showStates');
      | if strcmp(maskStr,'Hide (faster execution)')
      |   p=Simulink.Mask.get(gcb);
      |   autoCalcEn=get_param(gcb,'autoCalcEn');
      |   hintText=p.getDialogControl('timeHint');
      |   if strcmp(autoCalcEn,'on')
      |     param=p.getParameter('igain');
      |     if strcmp(param.Enabled,'off')
      |       SampleTime=Simulink.data.evalinGlobal(bdroot,get_param(gcb,'SampleTime'));
      |       if SampleTime==-1
      |         SampleTime=str2double(get_param(gcb,'SampleTime_1'));
      |         if isnan(SampleTime)
      |           hintText.Prompt=['Note: Implementation parameters cannot be calculated yet because the block''s inherited sample time is unknown. Simulink will update the sample time when you run the simulation.'];
      |         else
      |           hintText.Prompt=['Caution: Implementation parameters depend on inherited sample time. Make sure that the sample time of the block''s inputs corresponds to the sampling period in the target application.'];
      |         end
      |       else
      |         hintText.Prompt='Caution: Implementation parameters depend on the sample time. Make sure that the simulation time step corresponds to the sampling period in the target application.';
      |       end
      |       p=Simulink.Mask.get(gcb);
      |       param=p.getParameter('pgain');
      |       param.set('Enabled','on');
      |       param=p.getParameter('igain');
      |       param.set('Enabled','on');
      |     else
      |       SampleTime=Simulink.data.evalinGlobal(bdroot,get_param(gcb,'SampleTime'));
      |       if SampleTime==-1
      |         SampleTime=str2double(get_param(gcb,'SampleTime_1'));
      |       end
      |     end
      |     fltPropGain_bkup=get_param(gcb,'fltPropGain');
      |     fltIntegGain_bkup=get_param(gcb,'fltIntegGain');
      |     pgain=Simulink.data.evalinGlobal(bdroot,get_param(gcb,'pgain'));
      |     igain=Simulink.data.evalinGlobal(bdroot,get_param(gcb,'igain'));
      |     fltPropGain=pgain;
      |     fltIntegGain=igain*SampleTime*0.5;
      |     if isnan(fltPropGain)
      |       if ~strcmp(fltPropGain_bkup,'0')
      |         set_param(gcb,'fltPropGain','0');
      |       end
      |     else
      |       tmps=num2str(fltPropGain);
      |       if ~strcmp(fltPropGain_bkup,tmps)
      |         set_param(gcb,'fltPropGain',tmps);
      |       end
      |     end
      |     if isnan(fltIntegGain)
      |       if ~strcmp(fltIntegGain_bkup,'0')
      |         set_param(gcb,'fltIntegGain','0');
      |       end
      |     else
      |       tmps=num2str(fltIntegGain);
      |       if ~strcmp(fltIntegGain_bkup,tmps)
      |         set_param(gcb,'fltIntegGain',tmps);
      |       end
      |     end
      |   else
      |     param=p.getParameter('igain');
      |     if strcmp(param.Enabled,'on')
      |       hintText.Prompt='Caution: Implementation parameters are fixed.';
      |       p=Simulink.Mask.get(gcb);
      |       param=p.getParameter('pgain');
      |       param.set('Enabled','off');
      |       param=p.getParameter('igain');
      |       param.set('Enabled','off');
      |     end
      |   end
      | end
      mask DialogControl CompBut Prompt: Recalculate sample times
      mask DialogControl CompBut Tooltip: Simulink updates the sample times of all blocks when the simulation is run. This button will update the sample times now.
      mask DialogControl CompBut Callback:
      | btn=questdlg('This will apply all changes in all open dialog boxes and update the schematic. Do you want to proceed?','Apply all changes','Continue','Cancel','Continue');
      | if strcmp(btn,'Continue')
      |   dlgs=DAStudio.ToolRoot.getOpenDialogs;
      |   for i=1:length(dlgs)
      |     dlgs(i).apply;
      |   end
      |   try
      |     SampleTime_1=str2double(get_param(gcb,'SampleTime_1'));
      |     ts=Simulink.Block.getSampleTimes(gcb);
      |     ts=ts(1).Value(1);
      |     if (SampleTime_1 ~= ts)
      |       SampleTime_1=ts;
      |       set_param(gcb,'SampleTime_1',num2str(ts));
      |       autoCalcEn=get_param(gcb,'autoCalcEn');
      |       if strcmp(autoCalcEn,'on')
      |         SampleTime=Simulink.data.evalinGlobal(bdroot,get_param(gcb,'SampleTime'));
      |         p=Simulink.Mask.get(gcb);
      |         hintText=p.getDialogControl('timeHint');
      |         if SampleTime==-1
      |           SampleTime=SampleTime_1;
      |           hintText.Prompt='Caution: Implementation parameters depend on inherited sample time. Make sure that the sample time of the block''s inputs corresponds to the sampling period in the target application.';
      |         else
      |           hintText.Prompt='Caution: Implementation parameters depend on the sample time. Make sure that the simulation time step corresponds to the sampling period in the target application.';
      |         end
      |         fltPropGain_bkup=get_param(gcb,'fltPropGain');
      |         fltIntegGain_bkup=get_param(gcb,'fltIntegGain');
      |         pgain=Simulink.data.evalinGlobal(bdroot,get_param(gcb,'pgain'));
      |         igain=Simulink.data.evalinGlobal(bdroot,get_param(gcb,'igain'));
      |         fltPropGain=pgain;
      |         fltIntegGain=igain*SampleTime*0.5;
      |         if isnan(fltPropGain)
      |           if ~strcmp(fltPropGain_bkup,'0')
      |             set_param(gcb,'fltPropGain','0');
      |           end
      |         else
      |           tmps=num2str(fltPropGain);
      |           if ~strcmp(fltPropGain_bkup,tmps)
      |             set_param(gcb,'fltPropGain',tmps);
      |           end
      |         end
      |         if isnan(fltIntegGain)
      |           if ~strcmp(fltIntegGain_bkup,'0')
      |             set_param(gcb,'fltIntegGain','0');
      |           end
      |         else
      |           tmps=num2str(fltIntegGain);
      |           if ~strcmp(fltIntegGain_bkup,tmps)
      |             set_param(gcb,'fltIntegGain',tmps);
      |           end
      |         end
      |       end
      |     end
      |   catch
      |    warning(['Sample time cannot be calculated for the block ' gcb])
      |   end
      | end
      mask DialogControl timeHint Prompt: Note: Implementation parameters cannot be calculated yet because the block's inherited sample time is unknown. Simulink will update the sample time when you run the simulation.
      mask Display:
      | color('black');
      | pos = get_param(gcb, 'Position');
      | width = pos(3) - pos(1);
      | height = pos(4) - pos(2);
      | tX=width/2;
      | tY=height - 25;
      | color('black');
      | text(tX,tY, 'GFLIB_ControllerPIp_FLT', 'horizontalAlignment', 'center');
      | if showStates == 2
      |   color('red');
      |   text(tX,tY - 20, ['debugging mode' char(13) char(10) '(limited performance)'], 'horizontalAlignment', 'center');
      | end
  GFLIB_ControllerPIrAW_FLT : Subsystem  StartFcn=|  TreatAsAtomicUnit=on  mask(GFLIB_ControllerPIrAW_FLT){showStates=Hide (faster execution), resetStatesEnable=Pre-set according to the first set of inputs after reset, SampleTime=-1, intmethod=Trapezoidal, pgain=5, igain=0.5, upperLimit=10, lowerLimit=-10, autoCalcEn=on, fltUpperLimit=0, fltLowerLimit=0, fltCC1sc=0, fltCC2sc=0, SampleTime_1=NaN}
      | ts=get_param(gcb,'CompiledSampleTime');
      | if iscell(ts)
      |   ts=ts{1};
      |   if iscell(ts)
      |     ts=ts{1};
      |   end
      | end
      | ts=ts(1);
      | set_param(gcb,'SampleTime_1',num2str(ts));
      | p=Simulink.Mask.get(gcb);
      | hintText=p.getDialogControl('timeHint');
      | SampleTime=Simulink.data.evalinGlobal(bdroot,get_param(gcb,'SampleTime'));
      | p=Simulink.Mask.get(gcb);
      | autoCalcEn=get_param(gcb,'autoCalcEn');
      | if strcmp(autoCalcEn,'on')
      |   if SampleTime==-1
      |     hintText.Prompt='Caution: Implementation parameters depend on inherited sample time. Make sure that the sample time of the block''s inputs corresponds to the sampling period in the target application.';
      |   else
      |     hintText.Prompt='Caution: Implementation parameters depend on the sample time. Make sure that the simulation time step corresponds to the sampling period in the target application.';
      |   end
      |   SampleTime=ts;
      |   fltUpperLimit_bkup=get_param(gcb,'fltUpperLimit');
      |   fltLowerLimit_bkup=get_param(gcb,'fltLowerLimit');
      |   fltCC1sc_bkup=get_param(gcb,'fltCC1sc');
      |   fltCC2sc_bkup=get_param(gcb,'fltCC2sc');
      |   intmethod=get_param(gcb,'intmethod');
      |   pgain=Simulink.data.evalinGlobal(bdroot,get_param(gcb,'pgain'));
      |   igain=Simulink.data.evalinGlobal(bdroot,get_param(gcb,'igain'));
      |   upperLimit=Simulink.data.evalinGlobal(bdroot,get_param(gcb,'upperLimit'));
      |   lowerLimit=Simulink.data.evalinGlobal(bdroot,get_param(gcb,'lowerLimit'));
      |   if (upperLimit<=lowerLimit)
      |     warning('UpperLimit should be greater than LowerLimit.');
      |   end
      |   if strcmp(intmethod,'Forward Rectangular')
      |     cc1=pgain;
      |     cc2=-pgain+igain*SampleTime;
      |   else
      |     if strcmp(intmethod,'Backward Rectangular')
      |       cc1=pgain+igain*SampleTime;
      |       cc2=-pgain;
      |     else
      |       cc1=pgain+igain*SampleTime*0.5;
      |       cc2=-pgain+igain*SampleTime*0.5;
      |     end
      |   end
      |   fltCC1sc=cc1;
      |   fltCC2sc=cc2;
      |   fltUpperLimit=upperLimit;
      |   fltLowerLimit=lowerLimit;
      |   if isnan(fltUpperLimit)
      |     if ~strcmp(fltUpperLimit_bkup,'0')
      |       set_param(gcb,'fltUpperLimit','0');
      |     end
      |   else
      |     tmps=num2str(fltUpperLimit);
      |     if ~strcmp(fltUpperLimit_bkup,tmps)
      |       set_param(gcb,'fltUpperLimit',tmps);
      |     end
      |   end
      |   if isnan(fltLowerLimit)
      |     if ~strcmp(fltLowerLimit_bkup,'0')
      |       set_param(gcb,'fltLowerLimit','0');
      |     end
      |   else
      |     tmps=num2str(fltLowerLimit);
      |     if ~strcmp(fltLowerLimit_bkup,tmps)
      |       set_param(gcb,'fltLowerLimit',tmps);
      |     end
      |   end
      |   if isnan(fltCC1sc)
      |     if ~strcmp(fltCC1sc_bkup,'0')
      |       set_param(gcb,'fltCC1sc','0');
      |     end
      |   else
      |     tmps=num2str(fltCC1sc);
      |     if ~strcmp(fltCC1sc_bkup,tmps)
      |       set_param(gcb,'fltCC1sc',tmps);
      |     end
      |   end
      |   if isnan(fltCC2sc)
      |     if ~strcmp(fltCC2sc_bkup,'0')
      |       set_param(gcb,'fltCC2sc','0');
      |     end
      |   else
      |     tmps=num2str(fltCC2sc);
      |     if ~strcmp(fltCC2sc_bkup,tmps)
      |       set_param(gcb,'fltCC2sc',tmps);
      |     end
      |   end
      | end
      mask prompts: showStates "Show internal states:"; resetStatesEnable "Internal state after reset:"; SampleTime "Sample time (-1 for inherited):"; intmethod "Integration method:"; pgain "Proportional gain (P):"; igain "Integral gain (I):"; upperLimit "Controller upper limit:"; lowerLimit "Controller lower limit:"; autoCalcEn "Calculate implementation parameters from physical parameters"; fltUpperLimit "fltUpperLimit (Upper Limit of the controller):"; fltLowerLimit "fltLowerLimit (Lower Limit of the controller):"; fltCC1sc "fltCC1sc (CC1 coefficient):"; fltCC2sc "fltCC2sc (CC2 coefficient):"; SampleTime_1 "Discrete sample time:"
      mask help: Recurrent form discrete-time PI controller with anti-windup in single precision floating-point implementation. This block supports re-initialization of the internal state during simulation. If the block is reset, the controller's output will be aligned with the input fltControllerPIrAWOut_preset. Refer to the AMMCLIB User's Guide for further details.
      mask init:
      | ddName = get_param(bdroot,'DataDictionary');
      | if length(ddName)==0
      |   set_param(bdroot,'DataDictionary','ammclib_types.sldd');
      | else
      |   dd = Simulink.data.dictionary.open(ddName);
      |   data = getSection(dd,'Design Data');
      |   if ~exist(data,'SWLIBS_2Syst_F16')
      |     addDataSource(dd,'ammclib_types.sldd');
      |     saveChanges(dd);
      |   end
      | end
      | 
      | if showStates == 1
      |   % hidden state variables
      |   if strcmp(get_param([gcb '/fltUpperLimit'], 'BlockType'), 'Inport')
      |     posblk = get_param(gcb, 'Position');
      | 
      |     pos = get_param([gcb, '/fltUpperLimit'], 'Position');
      |     orient = get_param([gcb, '/fltUpperLimit'], 'Orientation');
      |     delete_block([gcb, '/fltUpperLimit']);
      |     add_block('built-in/Ground', [gcb, '/fltUpperLimit'], 'Position', pos, 'Orientation', orient);
      | 
      |     pos = get_param([gcb, '/fltLowerLimit'], 'Position');
      |     orient = get_param([gcb, '/fltLowerLimit'], 'Orientation');
      |     delete_block([gcb, '/fltLowerLimit']);
      |     add_block('built-in/Ground', [gcb, '/fltLowerLimit'], 'Position', pos, 'Orientation', orient);
      | 
      |     pos = get_param([gcb, '/fltAcc'], 'Position');
      |     orient = get_param([gcb, '/fltAcc'], 'Orientation');
      |     delete_block([gcb, '/fltAcc']);
      |     add_block('built-in/Ground', [gcb, '/fltAcc'], 'Position', pos, 'Orientation', orient);
      | 
      |     pos = get_param([gcb, '/fltInErrK1'], 'Position');
      |     orient = get_param([gcb, '/fltInErrK1'], 'Orientation');
      |     delete_block([gcb, '/fltInErrK1']);
      |     add_block('built-in/Ground', [gcb, '/fltInErrK1'], 'Position', pos, 'Orientation', orient);
      | 
      |     pos = get_param([gcb, '/fltCC1sc'], 'Position');
      |     orient = get_param([gcb, '/fltCC1sc'], 'Orientation');
      |     delete_block([gcb, '/fltCC1sc']);
      |     add_block('built-in/Ground', [gcb, '/fltCC1sc'], 'Position', pos, 'Orientation', orient);
      | 
      |     pos = get_param([gcb, '/fltCC2sc'], 'Position');
      |     orient = get_param([gcb, '/fltCC2sc'], 'Orientation');
      |     delete_block([gcb, '/fltCC2sc']);
      |     add_block('built-in/Ground', [gcb, '/fltCC2sc'], 'Position', pos, 'Orientation', orient);
      | 
      | 
      |     pmask=Simulink.Mask.get(gcb);
      |     pctrl=pmask.getParameter('SampleTime');
      |     pctrl.set('TypeOptions',{'fltInErr/SampleTime','fltControllerPIrAWOut_preset/SampleTime'});
      | 
      |     pos = get_param([gcb '/fltAcc_Out'], 'Position');
      |     orient = get_param([gcb '/fltAcc_Out'], 'Orientation');
      |     delete_block([gcb '/fltAcc_Out']);
      |     add_block('built-in/Terminator', [gcb '/fltAcc_Out'], 'Position', pos, 'Orientation', orient);
      | 
      |     pos = get_param([gcb '/fltInErrK1_Out'], 'Position');
      |     orient = get_param([gcb '/fltInErrK1_Out'], 'Orientation');
      |     delete_block([gcb '/fltInErrK1_Out']);
      |     add_block('built-in/Terminator', [gcb '/fltInErrK1_Out'], 'Position', pos, 'Orientation', orient);
      | 
      |     set_param([gcb '/fltInErr'], 'Port', '1');
      |     set_param([gcb '/fltControllerPIrAWOut_preset'], 'Port', '2');
      | 
      |     tmpOutCnt=0;
      |     tmpOutCnt=tmpOutCnt+1;
      |     set_param([gcb '/fltOut'], 'Port', num2str(tmpOutCnt));
      | 
      |     autoCalcEn=get_param(gcb,'autoCalcEn');
      |     if strcmp(autoCalcEn,'on')
      |       set_param(gcb,'MaskEnables',{'on','on','on','on','on','on','on','on','on','on','on','on','on','off'});
      |     else
      |       set_param(gcb,'MaskEnables',{'on','on','on','off','off','off','off','off','on','on','on','on','on','off'});
      |     end
      | 
      |     if (posblk(4) - posblk(2)) > 75
      |       height = 75;
      |       set_param(gcb,'Position',[posblk(1), posblk(2), posblk(3), posblk(2)+height])
      |     end
      |   end
      | else
      |   % shown state variables
      |   if strcmp(get_param([gcb '/fltUpperLimit'], 'BlockType'), 'Ground')
      |     posblk = get_param(gcb, 'Position');
      | 
      |     pos = get_param([gcb, '/fltUpperLimit'], 'Position');
      |     orient = get_param([gcb, '/fltUpperLimit'], 'Orientation');
      |     delete_block([gcb, '/fltUpperLimit']);
      |     add_block('built-in/Inport', [gcb, '/fltUpperLimit'], 'Position', pos, 'Orientation', orient, 'OutDataTypeStr', 'single');
      | 
      |     pos = get_param([gcb, '/fltLowerLimit'], 'Position');
      |     orient = get_param([gcb, '/fltLowerLimit'], 'Orientation');
      |     delete_block([gcb, '/fltLowerLimit']);
      |     add_block('built-in/Inport', [gcb, '/fltLowerLimit'], 'Position', pos, 'Orientation', orient, 'OutDataTypeStr', 'single');
      | 
      |     pos = get_param([gcb, '/fltAcc'], 'Position');
      |     orient = get_param([gcb, '/fltAcc'], 'Orientation');
      |     delete_block([gcb, '/fltAcc']);
      |     add_block('built-in/Inport', [gcb, '/fltAcc'], 'Position', pos, 'Orientation', orient, 'OutDataTypeStr', 'single');
      | 
      |     pos = get_param([gcb, '/fltInErrK1'], 'Position');
      |     orient = get_param([gcb, '/fltInErrK1'], 'Orientation');
      |     delete_block([gcb, '/fltInErrK1']);
      |     add_block('built-in/Inport', [gcb, '/fltInErrK1'], 'Position', pos, 'Orientation', orient, 'OutDataTypeStr', 'single');
      | 
      |     pos = get_param([gcb, '/fltCC1sc'], 'Position');
      |     orient = get_param([gcb, '/fltCC1sc'], 'Orientation');
      |     delete_block([gcb, '/fltCC1sc']);
      |     add_block('built-in/Inport', [gcb, '/fltCC1sc'], 'Position', pos, 'Orientation', orient, 'OutDataTypeStr', 'single');
      | 
      |     pos = get_param([gcb, '/fltCC2sc'], 'Position');
      |     orient = get_param([gcb, '/fltCC2sc'], 'Orientation');
      |     delete_block([gcb, '/fltCC2sc']);
      |     add_block('built-in/Inport', [gcb, '/fltCC2sc'], 'Position', pos, 'Orientation', orient, 'OutDataTypeStr', 'single');
      | 
      | 
      | 
      |     pos = get_param([gcb '/fltAcc_Out'], 'Position');
      |     orient = get_param([gcb '/fltAcc_Out'], 'Orientation');
      |     delete_block([gcb '/fltAcc_Out']);
      |     add_block('built-in/Outport', [gcb '/fltAcc_Out'], 'Position', pos, 'Orientation', orient);
      | 
      |     pos = get_param([gcb '/fltInErrK1_Out'], 'Position');
      |     orient = get_param([gcb '/fltInErrK1_Out'], 'Orientation');
      |     delete_block([gcb '/fltInErrK1_Out']);
      |     add_block('built-in/Outport', [gcb '/fltInErrK1_Out'], 'Position', pos, 'Orientation', orient);
      | 
      | 
      |     pmask=Simulink.Mask.get(gcb);
      |     pctrl=pmask.getParameter('SampleTime');
      |     pctrl.set('TypeOptions',{'fltInErr/SampleTime','fltControllerPIrAWOut_preset/SampleTime','fltUpperLimit/SampleTime','fltLowerLimit/SampleTime','fltAcc/SampleTime','fltInErrK1/SampleTime','fltCC1sc/SampleTime','fltCC2sc/SampleTime'});
      | 
      |     set_param([gcb '/fltInErr'], 'Port', '1');
      |     set_param([gcb '/fltControllerPIrAWOut_preset'], 'Port', '2');
      |     set_param([gcb '/fltUpperLimit'], 'Port', '3');
      |     set_param([gcb '/fltLowerLimit'], 'Port', '4');
      |     set_param([gcb '/fltAcc'], 'Port', '5');
      |     set_param([gcb '/fltInErrK1'], 'Port', '6');
      |     set_param([gcb '/fltCC1sc'], 'Port', '7');
      |     set_param([gcb '/fltCC2sc'], 'Port', '8');
      | 
      |     tmpOutCnt=0;
      |     tmpOutCnt=tmpOutCnt+1;
      |     set_param([gcb '/fltOut'], 'Port', num2str(tmpOutCnt));
      |     tmpOutCnt=tmpOutCnt+1;
      |     set_param([gcb '/fltAcc_Out'], 'Port', num2str(tmpOutCnt));
      |     tmpOutCnt=tmpOutCnt+1;
      |     set_param([gcb '/fltInErrK1_Out'], 'Port', num2str(tmpOutCnt));
      | 
      |     set_param(gcb,'MaskEnables',{'on','on','on','off','off','off','off','off','off','off','off','off','off','off'});
      | 
      |     if (posblk(4) - posblk(2)) < 225
      |       height = 225;
      |       set_param(gcb,'Position',[posblk(1), posblk(2), posblk(3), posblk(2)+height])
      |     end
      |   end
      | end
      settings: RTWSystemCode=Inline
      mask Help: web([fileparts(which('ammclib_bam_S32K3xx.slx')) '/../doc/S32K3XXMCLUG.pdf'], '-browser')
      mask TypeOptions showStates: Hide (faster execution) | Show (allows debugging; connect feedback loops manually)
      mask Callback showStates:
      | maskStr=get_param(gcb,'showStates');
      | if strcmp(maskStr,'Hide (faster execution)')
      |   if strcmp(get_param([gcb '/fltUpperLimit'], 'BlockType'), 'Inport')
      |     autoCalcEn=get_param(gcb,'autoCalcEn');
      |     if strcmp(autoCalcEn,'on')
      |       set_param(gcb,'MaskEnables',{'on','on','on','on','on','on','on','on','on','on','on','on','on','off'});
      |     else
      |       set_param(gcb,'MaskEnables',{'on','on','on','off','off','off','off','off','on','on','on','on','on','off'});
      |     end
      |   end
      | else
      |   if strcmp(get_param([gcb '/fltUpperLimit'], 'BlockType'), 'Ground')
      |     set_param(gcb,'MaskEnables',{'on','on','on','off','off','off','off','off','off','off','off','off','off','off'});
      |   end
      | end
      mask TypeOptions resetStatesEnable: Pre-set according to the first set of inputs after reset | Clear to zero
      mask TypeOptions SampleTime: fltInErr/SampleTime | fltControllerPIrAWOut_preset/SampleTime
      mask Callback SampleTime:
      | p=Simulink.Mask.get(gcb);
      | hintText=p.getDialogControl('timeHint');
      | SampleTime=Simulink.data.evalinGlobal(bdroot,get_param(gcb,'SampleTime'));
      | SampleTime_1=str2double(get_param(gcb,'SampleTime_1'));
      | if (((SampleTime==-1) && (~contains(hintText.Prompt,'inherited'))) || ...
      |     ((SampleTime~=-1) && contains(hintText.Prompt,'inherited')) || ...
      |     ((SampleTime~=-1) && (SampleTime_1~=SampleTime)) || ...
      |     ((SampleTime_1~=-1) && contains(hintText.Prompt,'yet')))
      |   if ((SampleTime==-1) && (~contains(hintText.Prompt,'inherited')))
      |     set_param(gcb,'SampleTime_1',num2str(NaN));
      |     SampleTime_1=NaN;
      |   end
      |   if (SampleTime~=-1)
      |     set_param(gcb,'SampleTime_1',num2str(SampleTime));
      |     SampleTime_1=SampleTime;
      |   end
      |   autoCalcEn=get_param(gcb,'autoCalcEn');
      |   if strcmp(autoCalcEn,'on')
      |     p=Simulink.Mask.get(gcb);
      |     hintText=p.getDialogControl('timeHint');
      |     if SampleTime==-1
